simulink model "PhaseII_opalrt_NoProtection"  (Simulink 8.8)
settings: Solver=ode3  StartTime=0.0  StopTime=inf  FixedStep=Ts  RelTol=1e-5  EnableMultiTasking=on
PostLoadFcn:
  | %BESS ctrl
  | Kpf=0.005*3*12;
  | Kif=5*6;
  | 
  | Kpf1=0.005*3*12;
  | Kif1=5*6;
  | Kp_v=0.016*15*35;
  | Ki_v=12*25;
  | 
  | Kp_v1=0.016*15*35;
  | Ki_v1=12*25;
  | 
  | Vabc_B=12.47e3;
  | Vdc_ref=Vabc_B*2;
  | Kpwm=sqrt(2)*Vabc_B/Vdc_ref;
  | ZB=Vabc_B^2/1e6;
  | R=0.005*ZB;
  | Ibasefull=673/2*sqrt(2);
  | 
  | 
  | Ts_Control=1e-4;
  | ts=0.05;
  | delay=0.2;
  | offset=10e3;
  | t_plan=60;
  | t_monitor=.2;
  | t_mon=t_monitor;
  | scalingfactor=1;
  | x=0.5;
  | n=6;
  | %t_plan=1/15;
  | %t_monitor=10/900;
  | %t_mon=10/900;
  | 
  | %t_plan=1/5;
  | %t_monitor=10/300;
  | %t_mon=10/300;
  | %scalingfactor=1/300;
  | 
  | f0=60;
  | 
  | Pabc_B=1e6;
  | Iabc_B=Pabc_B*sqrt(2/3)/Vabc_B;  % pk value
  | Imax_1=2.5;
  | Ptrans_B=Pabc_B*200;
  | 
  | Vdc_ref=Vabc_B*2;
  | 
  | ZB=Vabc_B^2/Pabc_B;
  | L=0.1*ZB/2/pi/60;
  | R=0.1*ZB;
  | C=1/(4*pi^2*(2e3)^2*L);
  | 
  | LL=0.005*ZB/2/pi/60;
  | RR=0.005*ZB;
  | 
  | RC=0.02;
  | 
  | %%% Initial SOC %%%%
  | SOC_ini_BESS1=0.5;
  | ... (+223 lines)
InitFcn:
  | %BESS ctrl
  | Kpf=0.005*3*12;
  | Kif=5*6;
  | 
  | Kpf1=0.005*3*12;
  | Kif1=5*6;
  | Kp_v=0.016*15*35;
  | Ki_v=12*25;
  | 
  | Kp_v1=0.016*15*35;
  | Ki_v1=12*25;
  | 
  | Vabc_B=12.47e3;
  | Vdc_ref=Vabc_B*2;
  | Kpwm=sqrt(2)*Vabc_B/Vdc_ref;
  | ZB=Vabc_B^2/1e6;
  | R=0.005*ZB;
  | Ibasefull=673/2*sqrt(2);
  | 
  | 
  | Ts_Control=1e-4;
  | ts=0.05;
  | delay=0.2;
  | offset=10e3;
  | t_plan=60;
  | t_monitor=.2;
  | t_mon=t_monitor;
  | scalingfactor=1;
  | x=0.5;
  | n=6;
  | %t_plan=1/15;
  | %t_monitor=10/900;
  | %t_mon=10/900;
  | 
  | %t_plan=1/5;
  | %t_monitor=10/300;
  | %t_mon=10/300;
  | %scalingfactor=1/300;
  | 
  | f0=60;
  | 
  | Pabc_B=1e6;
  | Iabc_B=Pabc_B*sqrt(2/3)/Vabc_B;  % pk value
  | Imax_1=2.5;
  | Ptrans_B=Pabc_B*200;
  | 
  | Vdc_ref=Vabc_B*2;
  | 
  | ZB=Vabc_B^2/Pabc_B;
  | L=0.1*ZB/2/pi/60;
  | R=0.1*ZB;
  | C=1/(4*pi^2*(2e3)^2*L);
  | 
  | LL=0.005*ZB/2/pi/60;
  | RR=0.005*ZB;
  | 
  | RC=0.02;
  | 
  | %%% Initial SOC %%%%
  | SOC_ini_BESS1=0.5;
  | ... (+223 lines)
undefined symbols (not defined in the file): D1, Delta, DiscIntNeverNeededParam, Left, PG2ref, type, V
libraries: powerlib x220, powerlib_meascontrol x82, dspstat3 x54, dsparch4 x43, dspswit3 x24, simulink x19, simulink_extras x12, powerlib_extras x11, ssn_lib x7, artemis x6, rtlab x5, rtio_generic_dnp3 x5
(part 2 of 9)

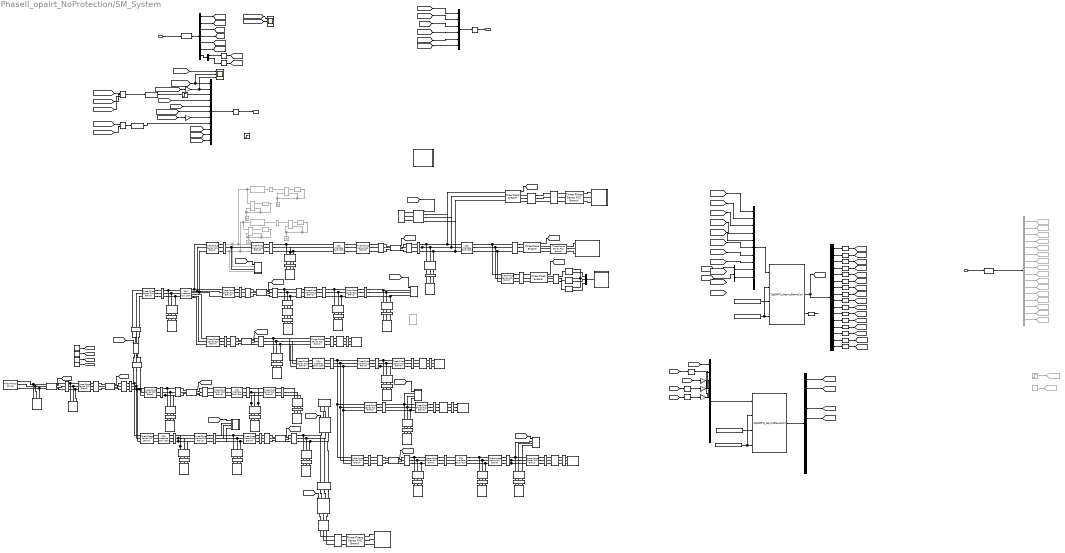
== system PhaseII_opalrt_NoProtection/SM_System ==
  note: DNP3 Communication
  note: Manual Control
  SC2SM : Inport
  SS2SM : Inport  Port=2
  2 kHz1 : dsparch4/Analog Filter Design  method=Butterworth  filttype=Lowpass  N=2  Wlo=2*pi*5  Whi=80  Rp=2  Rs=40
  2 kHz2 : dsparch4/Analog Filter Design  method=Butterworth  filttype=Lowpass  N=2  Wlo=2*pi*5  Whi=80  Rp=2  Rs=40
  2 kHz5 : dsparch4/Analog Filter Design  method=Butterworth  filttype=Lowpass  N=2  Wlo=2*pi*5  Whi=80  Rp=2  Rs=40
  Analog outputs init values1 : Constant  Value=0
  Analog outputs init values2 : Constant  Value=[0 0 0 0 0 0 0 0 0 0 0 0 0 0 0 0 0 0 0 0 0 0 0 0 0 0 0 0 0 0 0 0 0 0 0 0 0 0 0 0 0 0 0 0 0 0 0 0 0 0 0 0 0 0 0 ]
  Analog outputs init values3 : Constant  Value=[0 0 0 0 0 0 0 0 0 0 0 0 0 0 0 0 0 0 0 0 0 0 0 0 0 0 0 0 0 0 0 0 0 0 0 0 0 0 0 0 0 0 0 0 0 0 0 0 0 0 0 0 0 0 0 ]
  Analog outputs init values4 : Constant  Value=0
  Battery 2 : Subsystem  mask{eff=10, area=8e4}
      mask prompts: eff "Efficiency (%)"; area "Area (m^2)"
      mask help: The product of the effeciency, the area covered by the Pv farm and the irradiance in w/m2 will give you the power generate by the PV farm
      mask DialogControl DescGroupVar Prompt: PV farm
      mask DialogControl DescTextVar Prompt: The product of the efficiency, the area covered by the PV farm and the irradiance in W/m2 will give you the power generated by the PV farm.
      mask Display: image(imread('BESS.png'))
  "Battery 1 " : Subsystem  mask{eff=10, area=8e4}
      mask prompts: eff "Efficiency (%)"; area "Area (m^2)"
      mask help: The product of the effeciency, the area covered by the Pv farm and the irradiance in w/m2 will give you the power generate by the PV farm
      mask DialogControl DescGroupVar Prompt: PV farm
      mask DialogControl DescTextVar Prompt: The product of the efficiency, the area covered by the PV farm and the irradiance in W/m2 will give you the power generated by the PV farm.
      mask Display: image(imread('BESS.png'))
  Constant10 : Constant  Value=0.1
  Constant3 : Constant  Commented=on  Value=0.2
  Constant7 : Constant  Value=0.1
  Constant8 : Constant  Value=0.15
  Constant9 : Constant  Value=0.1
  Data Type Conversion{,1..18} (19 alike) : DataTypeConversion
  Demux : Demux  Outputs=3
  Demux13 : Demux  Outputs=16
  Demux14 : Demux  Outputs=10
  Demux17 : Demux  Outputs=2
  Demux2 : Demux  Outputs=[1 3 1 3 1 3 2]
  Demux3 : Demux  Commented=on  Outputs=[1 1 1 1 1 1 1 1 1 1 1 1 1 1 1 1]
  Distribution XFMR 010 : powerlib/Elements/Three-Phase Transformer (Two Windings)  Winding1Connection=Yg  Winding2Connection=Yg  CoreType=Three single-phase transformers  SetSaturation=off  Hysteresis=off  DataFile='hysteresis'  SetInitialFlux=off  Measurements=None  UNITS=pu  NominalPower=[ 750e3 , 60 ]  Winding1=[ 12.47e3 , 0.006*0.5 , 0.004*0.8 ]  Winding2=[ 120*sqrt(3) , 0.006 , 0.004*0.4 ]  Rm=339.61  Lm=332.223  L0=0.5  Saturation=[ 0,0 ; 0.0024,1.2 ; 1.0,1.52 ]  InitialFluxes=[-0.9942658300888 0.50146897071322 0.490639480643619]  MoreParameters=off  BreakLoop=on  DataType=off  TransfoNumber=1
  Distribution XFMR 011 : powerlib/Elements/Three-Phase Transformer (Two Windings)  Winding1Connection=Yg  Winding2Connection=Yg  CoreType=Three single-phase transformers  SetSaturation=off  Hysteresis=off  DataFile='hysteresis'  SetInitialFlux=off  Measurements=None  UNITS=pu  NominalPower=[ 750e3 , 60 ]  Winding1=[ 12.47e3 , 0.003*0.5 , 0.002*0.8 ]  Winding2=[ 120*sqrt(3) , 0.003 , 0.002*0.4 ]  Rm=391.76  Lm=422.949  L0=0.5  Saturation=[ 0,0 ; 0.0024,1.2 ; 1.0,1.52 ]  InitialFluxes=[-0.994208974756347 0.50135973621935 0.490459797609216]  MoreParameters=off  BreakLoop=on  DataType=off  TransfoNumber=1
  Distribution XFMR 012 : powerlib/Elements/Three-Phase Transformer (Two Windings)  Winding1Connection=Yg  Winding2Connection=Yg  CoreType=Three single-phase transformers  SetSaturation=off  Hysteresis=off  DataFile='hysteresis'  SetInitialFlux=off  Measurements=None  UNITS=pu  NominalPower=[ 750e3 , 60 ]  Winding1=[ 12.47e3 , 0.003*0.5 , 0.002*0.8 ]  Winding2=[ 120*sqrt(3) , 0.003 , 0.002*0.4 ]  Rm=391.76  Lm=422.949  L0=0.5  Saturation=[ 0,0 ; 0.0024,1.2 ; 1.0,1.52 ]  InitialFluxes=[-0.994702629209233 0.501353388807825 0.490097029757755]  MoreParameters=off  BreakLoop=on  DataType=off  TransfoNumber=1
  Distribution XFMR 013 : powerlib/Elements/Three-Phase Transformer (Two Windings)  Winding1Connection=Yg  Winding2Connection=Yg  CoreType=Three single-phase transformers  SetSaturation=off  Hysteresis=off  DataFile='hysteresis'  SetInitialFlux=off  Measurements=None  UNITS=pu  NominalPower=[ 750e3 , 60 ]  Winding1=[ 12.47e3 , 0.015*0.5 , 0.01*0.8 ]  Winding2=[ 120*sqrt(3) , 0.015 , 0.01*0.4 ]  Rm=391.76  Lm=422.949  L0=0.5  Saturation=[ 0,0 ; 0.0024,1.2 ; 1.0,1.52 ]  InitialFluxes=[-0.994614702520108 0.501538517038193 0.489928867290745]  MoreParameters=off  BreakLoop=on  DataType=off  TransfoNumber=1
  Distribution XFMR 014 : powerlib/Elements/Three-Phase Transformer (Two Windings)  Winding1Connection=Yg  Winding2Connection=Yg  CoreType=Three single-phase transformers  SetSaturation=off  Hysteresis=off  DataFile='hysteresis'  SetInitialFlux=off  Measurements=None  UNITS=pu  NominalPower=[ 750e3 , 60 ]  Winding1=[ 12.47e3 , 0.003*0.5 , 0.002*0.8 ]  Winding2=[ 120*sqrt(3) , 0.003 , 0.002*0.4 ]  Rm=391.76  Lm=422.949  L0=0.5  Saturation=[ 0,0 ; 0.0024,1.2 ; 1.0,1.52 ]  InitialFluxes=[-0.994115977169703 0.501412072072125 0.48984652002872]  MoreParameters=off  BreakLoop=on  DataType=off  TransfoNumber=1
  Distribution XFMR 02 : powerlib/Elements/Linear Transformer  Commented=on  UNITS=pu  NominalPower=[ 150e3 60 ]  winding1="[ 7.2e3  0.01  0.00667 ]"  winding2="[ 120  0.01  0.00667 ]"  ThreeWindings=off  winding3=[ 315e3 0.002 0.08 ]  RmLm=[ 318.75 327.548 ]  Measurements=None  DataType=off
  Distribution XFMR 03 : powerlib/Elements/Linear Transformer  Commented=on  UNITS=pu  NominalPower=[ 100e3 60 ]  winding1="[ 7.2e3  0.015  0.01 ]"  winding2="[ 120  0.015  0.01 ]"  ThreeWindings=off  winding3=[ 315e3 0.002 0.08 ]  RmLm=[ 308.32 322.496 ]  Measurements=None  DataType=off
  Distribution XFMR 04 : powerlib/Elements/Linear Transformer  Commented=on  UNITS=pu  NominalPower=[ 100e3 60 ]  winding1="[ 7.2e3  0.015  0.01 ]"  winding2="[ 120  0.015  0.01 ]"  ThreeWindings=off  winding3=[ 315e3 0.002 0.08 ]  RmLm=[ 308.32 322.496 ]  Measurements=None  DataType=off
  Distribution XFMR 05 : powerlib/Elements/Linear Transformer  Commented=on  UNITS=pu  NominalPower=[ 100e3 60 ]  winding1="[ 7.2e3  0.015  0.01 ]"  winding2="[ 120  0.015  0.01 ]"  ThreeWindings=off  winding3=[ 315e3 0.002 0.08 ]  RmLm=[ 308.32 322.496 ]  Measurements=None  DataType=off
  Distribution XFMR 06 : powerlib/Elements/Three-Phase Transformer (Two Windings)  Winding1Connection=Yg  Winding2Connection=Yg  CoreType=Three single-phase transformers  SetSaturation=off  Hysteresis=off  DataFile='hysteresis'  SetInitialFlux=off  Measurements=None  UNITS=pu  NominalPower=[ 725e3 , 60 ]  Winding1=[ 12.47e3 , 0.002*0.5 , 0.00133*0.8 ]  Winding2=[ 120*sqrt(3) , 0.002 , 0.00133*0.4 ]  Rm=443.91  Lm=376.523  L0=0.5  Saturation=[ 0,0 ; 0.0024,1.2 ; 1.0,1.52 ]  InitialFluxes=[-0.994629268867217 0.501113638204163 0.49204767683857]  MoreParameters=off  BreakLoop=on  DataType=off  TransfoNumber=1
  Distribution XFMR 07 : powerlib/Elements/Three-Phase Transformer (Two Windings)  Winding1Connection=Yg  Winding2Connection=Yg  CoreType=Three single-phase transformers  SetSaturation=off  Hysteresis=off  DataFile='hysteresis'  SetInitialFlux=off  Measurements=None  UNITS=pu  NominalPower=[ 900e3 , 60 ]  Winding1=[ 12.47e3 , 0.005*0.5 , 0.00333*0.8 ]  Winding2=[ 120*sqrt(3) , 0.005 , 0.00333*0.4 ]  Rm=350.04  Lm=312.414  L0=0.5  Saturation=[ 0,0 ; 0.0024,1.2 ; 1.0,1.52 ]  InitialFluxes=[-0.994045652632512 0.501511608393226 0.490384623138428]  MoreParameters=off  BreakLoop=on  DataType=off  TransfoNumber=1
  Distribution XFMR 08 : powerlib/Elements/Three-Phase Transformer (Two Windings)  Winding1Connection=Yg  Winding2Connection=Yg  CoreType=Three single-phase transformers  SetSaturation=off  Hysteresis=off  DataFile='hysteresis'  SetInitialFlux=off  Measurements=None  UNITS=pu  NominalPower=[ 750e3 , 60 ]  Winding1=[ 12.47e3 , 0.006*0.5 , 0.004*0.8 ]  Winding2=[ 120*sqrt(3) , 0.006 , 0.004*0.4 ]  Rm=339.61  Lm=332.223  L0=0.5  Saturation=[ 0,0 ; 0.0024,1.2 ; 1.0,1.52 ]  InitialFluxes=[-0.993941938198277 0.50151258800202 0.490279152869733]  MoreParameters=off  BreakLoop=on  DataType=off  TransfoNumber=1
  Distribution XFMR 09 : powerlib/Elements/Three-Phase Transformer (Two Windings)  Winding1Connection=Yg  Winding2Connection=Yg  CoreType=Three single-phase transformers  SetSaturation=off  Hysteresis=off  DataFile='hysteresis'  SetInitialFlux=off  Measurements=None  UNITS=pu  NominalPower=[ 750e3 , 60 ]  Winding1=[ 12.47e3 , 0.006*0.5 , 0.004*0.8 ]  Winding2=[ 120*sqrt(3) , 0.006 , 0.004*0.4 ]  Rm=339.61  Lm=332.223  L0=0.5  Saturation=[ 0,0 ; 0.0024,1.2 ; 1.0,1.52 ]  InitialFluxes=[-0.994119371539624 0.501403135186892 0.490542917279175]  MoreParameters=off  BreakLoop=on  DataType=off  TransfoNumber=1
  Distribution XFMR 1 : powerlib/Elements/Three-Phase Transformer (Two Windings)  Winding1Connection=Yg  Winding2Connection=Yg  CoreType=Three single-phase transformers  SetSaturation=off  Hysteresis=off  DataFile='hysteresis'  SetInitialFlux=off  Measurements=None  UNITS=pu  NominalPower=[ 812.5e3 , 60 ]  Winding1=[ 12.47e3 , 0.00089 , 0.00444 ]  Winding2=[ 480 , 0.00089 , 0.00444 ]  Rm=522.135  Lm=557.809  L0=0.5  Saturation=[ 0,0 ; 0.0024,1.2 ; 1.0,1.52 ]  InitialFluxes=[-0.995548930077736 0.501337560469489 0.493145095008447]  MoreParameters=off  BreakLoop=on  DataType=off  TransfoNumber=1
  Distribution XFMR 10 : powerlib/Elements/Three-Phase Transformer (Two Windings)  Winding1Connection=Yg  Winding2Connection=Yg  CoreType=Three single-phase transformers  SetSaturation=off  Hysteresis=off  DataFile='hysteresis'  SetInitialFlux=off  Measurements=None  UNITS=pu  NominalPower=[ 750e3 , 60 ]  Winding1=[ 12.47e3 , 0.00133 , 0.00667 ]  Winding2=[ 480 , 0.00133 , 0.00667 ]  Rm=443.91  Lm=404.751  L0=0.5  Saturation=[ 0,0 ; 0.0024,1.2 ; 1.0,1.52 ]  InitialFluxes=[-0.995768733272171 0.501268557544563 0.49352779195633]  MoreParameters=off  BreakLoop=on  DataType=off  TransfoNumber=1
  Distribution XFMR 11 : powerlib/Elements/Three-Phase Transformer (Two Windings)  Winding1Connection=Yg  Winding2Connection=Yg  CoreType=Three single-phase transformers  SetSaturation=off  Hysteresis=off  DataFile='hysteresis'  SetInitialFlux=off  Measurements=None  UNITS=pu  NominalPower=[ 750e3 , 60 ]  Winding1=[ 12.47e3 , 0.00133 , 0.00667 ]  Winding2=[ 480 , 0.00133 , 0.00667 ]  Rm=443.91  Lm=404.751  L0=0.5  Saturation=[ 0,0 ; 0.0024,1.2 ; 1.0,1.52 ]  InitialFluxes=[-0.994824104245158 0.501648177473995 0.492109909205201]  MoreParameters=off  BreakLoop=on  DataType=off  TransfoNumber=1
  Distribution XFMR 12 : powerlib/Elements/Three-Phase Transformer (Two Windings)  Winding1Connection=Yg  Winding2Connection=Yg  CoreType=Three single-phase transformers  SetSaturation=off  Hysteresis=off  DataFile='hysteresis'  SetInitialFlux=off  Measurements=None  UNITS=pu  NominalPower=[ 750e3 , 60 ]  Winding1=[ 12.47e3 , 0.00133 , 0.00667 ]  Winding2=[ 480 , 0.00133 , 0.00667 ]  Rm=443.91  Lm=404.751  L0=0.5  Saturation=[ 0,0 ; 0.0024,1.2 ; 1.0,1.52 ]  InitialFluxes=[-0.994885331973459 0.501617905967982 0.492199284760507]  MoreParameters=off  BreakLoop=on  DataType=off  TransfoNumber=1
  Distribution XFMR 14 : powerlib/Elements/Three-Phase Transformer (Two Windings)  Winding1Connection=Yg  Winding2Connection=Yg  CoreType=Three single-phase transformers  SetSaturation=off  Hysteresis=off  DataFile='hysteresis'  SetInitialFlux=off  Measurements=None  UNITS=pu  NominalPower=[ 812.5e3 , 60 ]  Winding1=[ 12.47e3 , 0.00089 , 0.00444 ]  Winding2=[ 480 , 0.00089 , 0.00444 ]  Rm=522.135  Lm=557.809  L0=0.5  Saturation=[ 0,0 ; 0.0024,1.2 ; 1.0,1.52 ]  InitialFluxes=[-0.995168363199261 0.501512793303796 0.492597007993423]  MoreParameters=off  BreakLoop=on  DataType=off  TransfoNumber=1
  Distribution XFMR 2 : powerlib/Elements/Three-Phase Transformer (Two Windings)  Winding1Connection=Yg  Winding2Connection=Yg  CoreType=Three single-phase transformers  SetSaturation=off  Hysteresis=off  DataFile='hysteresis'  SetInitialFlux=off  Measurements=None  UNITS=pu  NominalPower=[ 750e3 , 60 ]  Winding1=[ 12.47e3 , 0.00133 , 0.00667 ]  Winding2=[ 480 , 0.00133 , 0.00667 ]  Rm=443.91  Lm=404.751  L0=0.5  Saturation=[ 0,0 ; 0.0024,1.2 ; 1.0,1.52 ]  InitialFluxes=[-0.994824104245158 0.501648177473995 0.492109909205201]  MoreParameters=off  BreakLoop=on  DataType=off  TransfoNumber=1
  Distribution XFMR 3 : powerlib/Elements/Three-Phase Transformer (Two Windings)  Winding1Connection=Yg  Winding2Connection=Yg  CoreType=Three single-phase transformers  SetSaturation=off  Hysteresis=off  DataFile='hysteresis'  SetInitialFlux=off  Measurements=None  UNITS=pu  NominalPower=[ 750e3 , 60 ]  Winding1=[ 12.47e3 , 0.00133 , 0.00667 ]  Winding2=[ 480 , 0.00133 , 0.00667 ]  Rm=443.91  Lm=404.751  L0=0.5  Saturation=[ 0,0 ; 0.0024,1.2 ; 1.0,1.52 ]  InitialFluxes=[-0.995594239290872 0.501339764461854 0.493138938060875]  MoreParameters=off  BreakLoop=on  DataType=off  TransfoNumber=1
  Distribution XFMR 4 : powerlib/Elements/Three-Phase Transformer (Two Windings)  Winding1Connection=Yg  Winding2Connection=Yg  CoreType=Three single-phase transformers  SetSaturation=off  Hysteresis=off  DataFile='hysteresis'  SetInitialFlux=off  Measurements=None  UNITS=pu  NominalPower=[ 750e3 , 60 ]  Winding1=[ 12.47e3 , 0.00133 , 0.00667 ]  Winding2=[ 480 , 0.00133 , 0.00667 ]  Rm=443.91  Lm=404.751  L0=0.5  Saturation=[ 0,0 ; 0.0024,1.2 ; 1.0,1.52 ]  InitialFluxes=[-0.995008547006552 0.501540735777986 0.492046020226542]  MoreParameters=off  BreakLoop=on  DataType=off  TransfoNumber=1
  Distribution XFMR 5 : powerlib/Elements/Three-Phase Transformer (Two Windings)  Winding1Connection=Yg  Winding2Connection=Yg  CoreType=Three single-phase transformers  SetSaturation=off  Hysteresis=off  DataFile='hysteresis'  SetInitialFlux=off  Measurements=None  UNITS=pu  NominalPower=[ 750e3 , 60 ]  Winding1=[ 12.47e3 , 0.00222 , 0.01111 ]  Winding2=[ 480 , 0.00222 , 0.01111 ]  Rm=381.330  Lm=323.959  L0=0.5  Saturation=[ 0,0 ; 0.0024,1.2 ; 1.0,1.52 ]  InitialFluxes=[-0.995775345556504 0.501284393321602 0.493471561656197]  MoreParameters=off  BreakLoop=on  DataType=off  TransfoNumber=1
  Distribution XFMR 6 : powerlib/Elements/Three-Phase Transformer (Two Windings)  Winding1Connection=Yg  Winding2Connection=Yg  CoreType=Three single-phase transformers  SetSaturation=off  Hysteresis=off  DataFile='hysteresis'  SetInitialFlux=off  Measurements=None  UNITS=pu  NominalPower=[ 750e3 , 60 ]  Winding1=[ 12.47e3 , 0.00222 , 0.01111 ]  Winding2=[ 480 , 0.00222 , 0.01111 ]  Rm=381.330  Lm=323.959  L0=0.5  Saturation=[ 0,0 ; 0.0024,1.2 ; 1.0,1.52 ]  InitialFluxes=[-0.995636947856055 0.50134328812622 0.493423111787892]  MoreParameters=off  BreakLoop=on  DataType=off  TransfoNumber=1
  Distribution XFMR 7 : powerlib/Elements/Three-Phase Transformer (Two Windings)  Winding1Connection=Yg  Winding2Connection=Yg  CoreType=Three single-phase transformers  SetSaturation=off  Hysteresis=off  DataFile='hysteresis'  SetInitialFlux=off  Measurements=None  UNITS=pu  NominalPower=[ 750e3 , 60 ]  Winding1=[ 12.47e3 , 0.00111 , 0.00556 ]  Winding2=[ 480 , 0.00111 , 0.00556 ]  Rm=475.200  Lm=495.783  L0=0.5  Saturation=[ 0,0 ; 0.0024,1.2 ; 1.0,1.52 ]  InitialFluxes=[-0.995429112842175 0.501437040144372 0.492976191256826]  MoreParameters=off  BreakLoop=on  DataType=off  TransfoNumber=1
  Distribution XFMR 8 : powerlib/Elements/Three-Phase Transformer (Two Windings)  Winding1Connection=Yg  Winding2Connection=Yg  CoreType=Three single-phase transformers  SetSaturation=off  Hysteresis=off  DataFile='hysteresis'  SetInitialFlux=off  Measurements=None  UNITS=pu  NominalPower=[ 750e3 , 60 ]  Winding1=[ 12.47e3 , 0.00222 , 0.01111 ]  Winding2=[ 480 , 0.00222 , 0.01111 ]  Rm=381.330  Lm=323.959  L0=0.5  Saturation=[ 0,0 ; 0.0024,1.2 ; 1.0,1.52 ]  InitialFluxes=[0.493153694918364 0.501391810391627 -0.995533055661482]  MoreParameters=off  BreakLoop=on  DataType=off  TransfoNumber=1
  Distribution XFMR 9 : powerlib/Elements/Three-Phase Transformer (Two Windings)  Winding1Connection=Yg  Winding2Connection=Yg  CoreType=Three single-phase transformers  SetSaturation=off  Hysteresis=off  DataFile='hysteresis'  SetInitialFlux=off  Measurements=None  UNITS=pu  NominalPower=[ 750e3 , 60 ]  Winding1=[ 12.47e3 , 0.00133 , 0.00667 ]  Winding2=[ 480 , 0.00133 , 0.00667 ]  Rm=443.91  Lm=404.751  L0=0.5  Saturation=[ 0,0 ; 0.0024,1.2 ; 1.0,1.52 ]  InitialFluxes=[-0.995385675641374 0.501454453441104 0.492920662481959]  MoreParameters=off  BreakLoop=on  DataType=off  TransfoNumber=1
  Gain2 : Gain  Gain=Pb/1e6
  Gain3 : Gain
  Gain4 : Gain  Gain=Pb/1e6
  Gain5 : Gain
  Gain6 : Gain  Gain=60
  Gen bus : powerlib/Measurements/Three-Phase V-I Measurement  VoltageMeasurement=phase-to-phase  SetLabelV=on  LabelV=VabcGen  Vpu=off  VpuLL=off  CurrentMeasurement=yes  SetLabelI=on  LabelI=IabcGen  Ipu=off  Pbase=Pb  Vbase=Vb*sqrt(3/2)  OutputType=Complex  PhasorSimulation=off  PSBequivalent=0
  Gen bus1 : powerlib/Measurements/Three-Phase V-I Measurement  VoltageMeasurement=phase-to-phase  SetLabelV=on  LabelV=VabcGen_internal  Vpu=off  VpuLL=off  CurrentMeasurement=yes  SetLabelI=on  LabelI=IabcGen_internal  Ipu=off  Pbase=Pb  Vbase=Vb*sqrt(3/2)  OutputType=Complex  PhasorSimulation=off  PSBequivalent=0
  Generator2 : Subsystem
  Goto1 : Goto  Commented=on  GotoTag=F3  TagVisibility=global
  Goto58 : Goto  Commented=on  GotoTag=S_Y3  TagVisibility=global
  Goto59 : Goto  Commented=on  GotoTag=S_Y4  TagVisibility=global
  Goto66 : Goto  Commented=on  GotoTag=S_Y5  TagVisibility=global
  Goto67 : Goto  Commented=on  GotoTag=S_Y6  TagVisibility=global
  Goto70 : Goto  Commented=on  GotoTag=G1_En  TagVisibility=global
  Goto72 : Goto  Commented=on  GotoTag=Grid_enable  TagVisibility=global
  Goto73 : Goto  Commented=on  GotoTag=S_G1  TagVisibility=global
  Goto74 : Goto  Commented=on  GotoTag=S_Y7  TagVisibility=global
  Goto75 : Goto  Commented=on  GotoTag=S_Y1  TagVisibility=global
  Goto76 : Goto  Commented=on  GotoTag=S_Y2  TagVisibility=global
  Goto77 : Goto  Commented=on  GotoTag=S_G2  TagVisibility=global
  Goto78 : Goto  Commented=on  GotoTag=S_Y8  TagVisibility=global
  Goto79 : Goto  Commented=on  GotoTag=F6  TagVisibility=global
  Goto80 : Goto  Commented=on  GotoTag=F7  TagVisibility=global
  Goto81 : Goto  Commented=on  GotoTag=Manual_Reset  TagVisibility=global
  Goto82 : Goto  Commented=on  GotoTag=Gen_P  TagVisibility=global
  Goto9 : Goto  Commented=on  GotoTag=F5  TagVisibility=global
  Ground{,2..4} (4 alike) : powerlib/Elements/Ground  Commented=on  LConnTagsString=a
  Intellirupter : Subsystem
  Load 1 : powerlib/Elements/Three-Phase Series RLC Load  LConnTagsString=A|B|C  Configuration=Y (grounded)  NominalVoltage=480  Vabc=[ 0.987168 0.986064 0.986504]*277.128  Vabcp=[1e3 1e3 1e3]  NominalFrequency=60  UnbalancedPower=on  ActivePower=10e3  InductivePower=100  CapacitivePower=100  Pabc=[17027.7904 21000.1348 17507.4994]*load_scale  QLabc=[11009.6057 13611.7741 11303.4274]*load_scale/10  QCabc=[0 0 0]  Pabcp=[10e3 9e3 11e3]  QLabcp=[100 90 110]  QCabcp=[100 90 110]  Measurements=None  LoadType=constant PQ
  Load 10 : powerlib/Elements/Three-Phase Series RLC Load  LConnTagsString=A|B|C  Configuration=Y (grounded)  NominalVoltage=480  Vabc=[ 0.994007 0.993686 0.993644]*277.128  Vabcp=[1e3 1e3 1e3]  NominalFrequency=60  UnbalancedPower=on  ActivePower=10e3  InductivePower=100  CapacitivePower=100  Pabc=[39119.69 48245.7642 40221.7746]*load_scale/2  QLabc=[25293.4968 31271.7251 25968.5235]*load_scale/2/10  QCabc=[0 0 0]  Pabcp=[10e3 9e3 11e3]  QLabcp=[100 90 110]  QCabcp=[100 90 110]  Measurements=None  LoadType=constant PQ
  Load 11 : powerlib/Elements/Three-Phase Series RLC Load  LConnTagsString=A|B|C  Configuration=Y (grounded)  NominalVoltage=480  Vabc=[ 0.992968 0.992478 0.992611]*277.128  Vabcp=[1e3 1e3 1e3]  NominalFrequency=60  UnbalancedPower=on  ActivePower=10e3  InductivePower=100  CapacitivePower=100  Pabc=[46970.1648 57927.6445 48293.4139]*load_scale  QLabc=[30369.354 37547.2833 31179.8439]*load_scale/10  QCabc=[0 0 0]  Pabcp=[10e3 9e3 11e3]  QLabcp=[100 90 110]  QCabcp=[100 90 110]  Measurements=None  LoadType=constant PQ
  Load 12 : powerlib/Elements/Three-Phase Series RLC Load  LConnTagsString=A|B|C  Configuration=Y (grounded)  NominalVoltage=480  Vabc=[ 0.993588 0.993244 0.993249]*277.128  Vabcp=[1e3 1e3 1e3]  NominalFrequency=60  UnbalancedPower=on  ActivePower=10e3  InductivePower=100  CapacitivePower=100  Pabc=[40129.5633 49491.2267 41260.0981]*load_scale  QLabc=[25946.4474 32079.0035 26638.8999]*load_scale/10  QCabc=[0 0 0]  Pabcp=[10e3 9e3 11e3]  QLabcp=[100 90 110]  QCabcp=[100 90 110]  Measurements=None  LoadType=constant PQ
  Load 13 : powerlib/Elements/Three-Phase Series RLC Load  LConnTagsString=A|B|C  Configuration=Y (grounded)  NominalVoltage=480  Vabc=[ 0.992901 0.992425 0.992496]*277.128  Vabcp=[1e3 1e3 1e3]  NominalFrequency=60  UnbalancedPower=on  ActivePower=10e3  InductivePower=100  CapacitivePower=100  Pabc=[1 1 1]  QLabc=[0 0 0]  QCabc=[0 0 0]  Pabcp=[10e3 9e3 11e3]  QLabcp=[100 90 110]  QCabcp=[100 90 110]  Measurements=None  LoadType=constant PQ
  Load 14 : powerlib/Elements/Three-Phase Series RLC Load  LConnTagsString=A|B|C  Configuration=Y (grounded)  NominalVoltage=480  Vabc=[ 0.992968 0.992478 0.992611]*277.128  Vabcp=[1e3 1e3 1e3]  NominalFrequency=60  UnbalancedPower=on  ActivePower=10e3  InductivePower=100  CapacitivePower=100  Pabc=[46970.1648 57927.6445 48293.4139]*load_scale  QLabc=[30369.354 37547.2833 31179.8439]*load_scale/10  QCabc=[0 0 0]  Pabcp=[10e3 9e3 11e3]  QLabcp=[100 90 110]  QCabcp=[100 90 110]  Measurements=None  LoadType=constant PQ
  Load 15 : powerlib/Elements/Three-Phase Series RLC Load  LConnTagsString=A|B|C  Configuration=Y (grounded)  NominalVoltage=480  Vabc=[ 0.992901 0.992425 0.992496]*277.128  Vabcp=[1e3 1e3 1e3]  NominalFrequency=60  UnbalancedPower=on  ActivePower=10e3  InductivePower=100  CapacitivePower=100  Pabc=[1 1 1]  QLabc=[0 0 0]  QCabc=[0 0 0]  Pabcp=[10e3 9e3 11e3]  QLabcp=[100 90 110]  QCabcp=[100 90 110]  Measurements=None  LoadType=constant PQ
  Load 2 : powerlib/Elements/Three-Phase Series RLC Load  LConnTagsString=A|B|C  Configuration=Y (grounded)  NominalVoltage=480  Vabc=[ 0.994058 0.994595 0.993585]*277.128  Vabcp=[1e3 1e3 1e3]  NominalFrequency=60  UnbalancedPower=on  ActivePower=10e3  InductivePower=100  CapacitivePower=100  Pabc=[81043.4347 89864.2131 82168.4451]*load_scale  QLabc=[52061.1336 58247.7865 53085.0614]*load_scale/10  QCabc=[0 0 0]  Pabcp=[10e3 9e3 11e3]  QLabcp=[100 90 110]  QCabcp=[100 90 110]  Measurements=None  LoadType=constant PQ
  Load 3 : powerlib/Elements/Three-Phase Series RLC Load  LConnTagsString=A|B|C  Configuration=Y (grounded)  NominalVoltage=480  Vabc=[ 0.992901 0.992425 0.992496]*277.128  Vabcp=[1e3 1e3 1e3]  NominalFrequency=60  UnbalancedPower=on  ActivePower=10e3  InductivePower=100  CapacitivePower=100  Pabc=[49962.928 61618.5773 51370.4895]*load_scale/2  QLabc=[32304.3756 39939.6557 33166.5069]*load_scale/2/10  QCabc=[0 0 0]  Pabcp=[10e3 9e3 11e3]  QLabcp=[100 90 110]  QCabcp=[100 90 110]  Measurements=None  LoadType=constant PQ
  Load 4 : powerlib/Elements/Three-Phase Series RLC Load  LConnTagsString=A|B|C  Configuration=Y (grounded)  NominalVoltage=480  Vabc=[ 0.99408 0.993727 0.99369]*277.128  Vabcp=[1e3 1e3 1e3]  NominalFrequency=60  UnbalancedPower=on  ActivePower=10e3  InductivePower=100  CapacitivePower=100  Pabc=[35013.8548 43182.0953 36000.2693]*load_scale/2  QLabc=[22638.7997 27989.5787 23242.9784]*load_scale/10  QCabc=[0 0 0]  Pabcp=[10e3 9e3 11e3]  QLabcp=[100 90 110]  QCabcp=[100 90 110]  Measurements=None  LoadType=constant PQ
  Load 5 : powerlib/Elements/Three-Phase Series RLC Load  LConnTagsString=A|B|C  Configuration=Y (grounded)  NominalVoltage=480  Vabc=[ 0.990244 0.989037 0.989784]*277.128  Vabcp=[1e3 1e3 1e3]  NominalFrequency=60  UnbalancedPower=on  ActivePower=10e3  InductivePower=100  CapacitivePower=100  Pabc=[28836.6737 35563.8646 29649.0639]*load_scale/2  QLabc=[18644.8388 23051.6278 19142.4277]*load_scale/2/10  QCabc=[0 0 0]  Pabcp=[10e3 9e3 11e3]  QLabcp=[100 90 110]  QCabcp=[100 90 110]  Measurements=None  LoadType=constant PQ
  Load 6 : powerlib/Elements/Three-Phase Series RLC Load  LConnTagsString=A|B|C  Configuration=Y (grounded)  NominalVoltage=480  Vabc=[ 0.989951 0.988653 0.989471]*277.128  Vabcp=[1e3 1e3 1e3]  NominalFrequency=60  UnbalancedPower=on  ActivePower=10e3  InductivePower=100  CapacitivePower=100  Pabc=[29787.5763 36736.5994 30626.7554]*load_scale/2  QLabc=[19259.6609 23811.7658 19773.6581]*load_scale/2/10  QCabc=[0 0 0]  Pabcp=[10e3 9e3 11e3]  QLabcp=[100 90 110]  QCabcp=[100 90 110]  Measurements=None  LoadType=constant PQ
  Load 7 : powerlib/Elements/Three-Phase Series RLC Load  LConnTagsString=A|B|C  Configuration=Y (grounded)  NominalVoltage=480  Vabc=[ 0.993519 0.993097 0.993157]*277.128  Vabcp=[1e3 1e3 1e3]  NominalFrequency=60  UnbalancedPower=on  ActivePower=10e3  InductivePower=100  CapacitivePower=100  Pabc=[64484.4635 79527.7832 66301.1275]*load_scale  QLabc=[41693.5199 51547.9652 42806.2264]*load_scale/10  QCabc=[0 0 0]  Pabcp=[10e3 9e3 11e3]  QLabcp=[100 90 110]  QCabcp=[100 90 110]  Measurements=None  LoadType=constant PQ
  Load 8 : powerlib/Elements/Three-Phase Series RLC Load  LConnTagsString=A|B|C  Configuration=Y (grounded)  NominalVoltage=480  Vabc=[ 0.991121 0.990439 0.991202]*277.128  Vabcp=[1e3 1e3 1e3]  NominalFrequency=60  UnbalancedPower=on  ActivePower=10e3  InductivePower=100  CapacitivePower=100  Pabc=[24399.1283 30091.1022 25086.5034]*load_scale  QLabc=[15775.6688 19504.317 16196.686]*load_scale/10  QCabc=[0 0 0]  Pabcp=[10e3 9e3 11e3]  QLabcp=[100 90 110]  QCabcp=[100 90 110]  Measurements=None  LoadType=constant PQ
  Load 9 : powerlib/Elements/Three-Phase Series RLC Load  LConnTagsString=A|B|C  Configuration=Y (grounded)  NominalVoltage=480  Vabc=[ 0.992758 0.992152 0.992379]*277.128  Vabcp=[1e3 1e3 1e3]  NominalFrequency=60  UnbalancedPower=on  ActivePower=10e3  InductivePower=100  CapacitivePower=100  Pabc=[52815.6357 65136.7817 54303.5641]*load_scale  QLabc=[34148.842 42220.0698 35060.198]*load_scale/10  QCabc=[0 0 0]  Pabcp=[10e3 9e3 11e3]  QLabcp=[100 90 110]  QCabcp=[100 90 110]  Measurements=None  LoadType=constant PQ
  Load Flow Bus : powerlib/Measurements/Load Flow Bus  LConnTagsString=a|b|c  RConnTagsString=a|b|c  Phases=ABC  Connectors=on both sides  ID=BUS_1  Vbase=7.2e3  Vref=[1 1 1]  Vangle=[0 -120 120]  VLF=1  VLFb=1  VLFc=1  angleLF=0  angleLFb=-120  angleLFc=120
  Load Flow Bus20 : powerlib/Measurements/Load Flow Bus  LConnTagsString=a|b|c  RConnTagsString=a|b|c  Phases=ABC  Connectors=on both sides  ID=BUS_2  Vbase=7.2e3  Vref=[1 1 1]  Vangle=[0 -120 120]  VLF=0.9976  VLFb=0.9981  VLFc=0.9973  angleLF=-0.1269  angleLFb=-120.1  angleLFc=119.9
  Load Flow Bus21 : powerlib/Measurements/Load Flow Bus  LConnTagsString=a|b|c  RConnTagsString=a|b|c  Phases=ABC  Connectors=on both sides  ID=BUS_11  Vbase=7.2e3  Vref=[1 1 1]  Vangle=[0 -120 120]  VLF=0.9972  VLFb=0.9977  VLFc=0.997  angleLF=-0.1433  angleLFb=-120.1  angleLFc=119.9
  Load Flow Bus22 : powerlib/Measurements/Load Flow Bus  LConnTagsString=a|b|c  RConnTagsString=a|b|c  Phases=ABC  Connectors=on both sides  ID=BUS_12  Vbase=7.2e3  Vref=[1 1 1]  Vangle=[0 -120 120]  VLF=0.9972  VLFb=0.9977  VLFc=0.997  angleLF=-0.1436  angleLFb=-120.1  angleLFc=119.9
  Load Flow Bus23 : powerlib/Measurements/Load Flow Bus  LConnTagsString=a|b|c  RConnTagsString=a|b|c  Phases=ABC  Connectors=on both sides  ID=BUS_3_0  Vbase=480/sqrt(3)  Vref=[1 1 1]  Vangle=[0 -120 120]  VLF=0.9935  VLFb=0.9931  VLFc=0.9932  angleLF=-0.3687  angleLFb=-120.4  angleLFc=119.6
  Load Flow Bus24 : powerlib/Measurements/Load Flow Bus  LConnTagsString=a|b|c  RConnTagsString=a|b|c  Phases=ABC  Connectors=on both sides  ID=BUS_4_0  Vbase=480/sqrt(3)  Vref=[1 1 1]  Vangle=[0 -120 120]  VLF=0.9911  VLFb=0.9904  VLFc=0.9912  angleLF=119.5  angleLFb=-120.6  angleLFc=-0.5043
  Load Flow Bus25 : powerlib/Measurements/Load Flow Bus  LConnTagsString=a|b|c  RConnTagsString=a|b|c  Phases=ABC  Connectors=on both sides  ID=BUS_5_0  Vbase=480/sqrt(3)  Vref=[1 1 1]  Vangle=[0 -120 120]  VLF=0.9928  VLFb=0.9922  VLFc=0.9924  angleLF=-0.413  angleLFb=-120.5  angleLFc=119.6
  Load Flow Bus26 : powerlib/Measurements/Load Flow Bus  LConnTagsString=a|b|c  RConnTagsString=a|b|c  Phases=ABC  Connectors=on both sides  ID=BUS_6_0  Vbase=480/sqrt(3)  Vref=[1 1 1]  Vangle=[0 -120 120]  VLF=0.9902  VLFb=0.989  VLFc=0.9898  angleLF=-0.5603  angleLFb=-120.6  angleLFc=119.4
  Load Flow Bus27 : powerlib/Measurements/Load Flow Bus  LConnTagsString=a|b|c  RConnTagsString=a|b|c  Phases=ABC  Connectors=on both sides  ID=BUS_7_0  Vbase=480/sqrt(3)  Vref=[1 1 1]  Vangle=[0 -120 120]  VLF=0.994  VLFb=0.9937  VLFc=0.9936  angleLF=-0.3395  angleLFb=-120.4  angleLFc=119.7
  Load Flow Bus28 : powerlib/Measurements/Load Flow Bus  LConnTagsString=a|b|c  RConnTagsString=a|b|c  Phases=ABC  Connectors=on both sides  ID=BUS_8_0  Vbase=480/sqrt(3)  Vref=[1 1 1]  Vangle=[0 -120 120]  VLF=0.99  VLFb=0.9887  VLFc=0.9895  angleLF=-0.5766  angleLFb=-120.7  angleLFc=119.4
  Load Flow Bus29 : powerlib/Measurements/Load Flow Bus  LConnTagsString=a|b|c  RConnTagsString=a|b|c  Phases=ABC  Connectors=on both sides  ID=BUS_9_0  Vbase=480/sqrt(3)  Vref=[1 1 1]  Vangle=[0 -120 120]  VLF=0.9929  VLFb=0.9924  VLFc=0.9925  angleLF=-0.4047  angleLFb=-120.4  angleLFc=119.6
  Load Flow Bus30 : powerlib/Measurements/Load Flow Bus  LConnTagsString=a|b|c  RConnTagsString=a|b|c  Phases=ABC  Connectors=on both sides  ID=BUS_10_0  Vbase=120  Vref=[1 1 1]  Vangle=[0 -120 120]  VLF=0.9855  VLFb=0.9834  VLFc=0.985  angleLF=-0.08438  angleLFb=-120  angleLFc=119.9
  Load Flow Bus31 : powerlib/Measurements/Load Flow Bus  LConnTagsString=a|b|c  RConnTagsString=a|b|c  Phases=ABC  Connectors=on both sides  ID=BUS_3  Vbase=7.2e3  Vref=[1 1 1]  Vangle=[0 -120 120]  VLF=0.9976  VLFb=0.9981  VLFc=0.9973  angleLF=-0.1275  angleLFb=-120.1  angleLFc=119.9
  Load Flow Bus32 : powerlib/Measurements/Load Flow Bus  LConnTagsString=a|b|c  RConnTagsString=a|b|c  Phases=ABC  Connectors=on both sides  ID=BUS_11_0  Vbase=480/sqrt(3)  Vref=[1 1 1]  Vangle=[0 -120 120]  VLF=0.993  VLFb=0.9925  VLFc=0.9926  angleLF=-0.3966  angleLFb=-120.4  angleLFc=119.6
  Load Flow Bus33 : powerlib/Measurements/Load Flow Bus  LConnTagsString=a|b|c  RConnTagsString=a|b|c  Phases=ABC  Connectors=on both sides  ID=BUS_12_0  Vbase=480/sqrt(3)  Vref=[1 1 1]  Vangle=[0 -120 120]  VLF=0.9936  VLFb=0.9932  VLFc=0.9932  angleLF=-0.3599  angleLFb=-120.4  angleLFc=119.6
  Load Flow Bus36 : powerlib/Measurements/Load Flow Bus  LConnTagsString=a|b|c  RConnTagsString=a|b|c  Phases=ABC  Connectors=on both sides  ID=BUS_13  Vbase=7.2e3  Vref=[1 1 1]  Vangle=[0 -120 120]  VLF=0.997  VLFb=0.9982  VLFc=0.9966  angleLF=-0.1665  angleLFb=-120.1  angleLFc=119.9
  Load Flow Bus37 : powerlib/Measurements/Load Flow Bus  LConnTagsString=a|b|c  RConnTagsString=a|b|c  Phases=ABC  Connectors=on both sides  ID=BUS_14  Vbase=7.2e3  Vref=[1 1 1]  Vangle=[0 -120 120]  VLF=0.997  VLFb=0.9982  VLFc=0.9966  angleLF=-0.1669  angleLFb=-120.1  angleLFc=119.9
  Load Flow Bus38 : powerlib/Measurements/Load Flow Bus  LConnTagsString=a|b|c  RConnTagsString=a|b|c  Phases=ABC  Connectors=on both sides  ID=BUS_15  Vbase=7.2e3  Vref=[1 1 1]  Vangle=[0 -120 120]  VLF=0.9969  VLFb=0.9982  VLFc=0.9966  angleLF=-0.167  angleLFb=-120.1  angleLFc=119.9
  Load Flow Bus39 : powerlib/Measurements/Load Flow Bus  LConnTagsString=a|b|c  RConnTagsString=a|b|c  Phases=ABC  Connectors=on both sides  ID=BUS_14_0  Vbase=480/sqrt(3)  Vref=[1 1 1]  Vangle=[0 -120 120]  VLF=0.9941  VLFb=0.9946  VLFc=0.9936  angleLF=-0.341  angleLFb=-120.3  angleLFc=119.7
  Load Flow Bus40 : powerlib/Measurements/Load Flow Bus  LConnTagsString=a|b|c  RConnTagsString=a|b|c  Phases=ABC  Connectors=on both sides  ID=BUS_15_0  Vbase=480/sqrt(3)  Vref=[1 1 1]  Vangle=[0 -120 120]  VLF=0.9872  VLFb=0.9861  VLFc=0.9865  angleLF=-0.746  angleLFb=-120.8  angleLFc=119.3
  Load Flow Bus41 : powerlib/Measurements/Load Flow Bus  Commented=on  LConnTagsString=a  RConnTagsString=a  Phases=A  Connectors=on both sides  ID=BUS_27  Vbase=7.2e3  Vref=1  Vangle=0  VLF=0.9964  VLFb=NaN  VLFc=NaN  angleLF=-0.1708  angleLFb=NaN  angleLFc=NaN
  Load Flow Bus42 : powerlib/Measurements/Load Flow Bus  Commented=on  LConnTagsString=a  RConnTagsString=a  Phases=C  Connectors=on both sides  ID=BUS_28  Vbase=7.2e3  Vref=1  Vangle=120  VLF=NaN  VLFb=NaN  VLFc=0.9958  angleLF=NaN  angleLFb=NaN  angleLFc=119.9
      settings: AttributesFormatString=|
      | %<ID>
      | %<Vbase>V
      | %<VLFc>pu
      | %<angleLFc>deg.
  Load Flow Bus43 : powerlib/Measurements/Load Flow Bus  LConnTagsString=a|b|c  RConnTagsString=a|b|c  Phases=ABC  Connectors=on both sides  ID=BUS_16  Vbase=7.2e3  Vref=[1 1 1]  Vangle=[0 -120 120]  VLF=0.9972  VLFb=0.9976  VLFc=0.9969  angleLF=-0.1422  angleLFb=-120.1  angleLFc=119.9
  Load Flow Bus44 : powerlib/Measurements/Load Flow Bus  LConnTagsString=a|b|c  RConnTagsString=a|b|c  Phases=ABC  Connectors=on both sides  ID=BUS_4  Vbase=7.2e3  Vref=[1 1 1]  Vangle=[0 -120 120]  VLF=0.9975  VLFb=0.9981  VLFc=0.9973  angleLF=-0.1279  angleLFb=-120.1  angleLFc=119.9
  Load Flow Bus45 : powerlib/Measurements/Load Flow Bus  LConnTagsString=a|b|c  RConnTagsString=a|b|c  Phases=ABC  Connectors=on both sides  ID=BUS_16_0  Vbase=480/sqrt(3)  Vref=[1 1 1]  Vangle=[0 -120 120]  VLF=0.9941  VLFb=0.9937  VLFc=0.9937  angleLF=-0.331  angleLFb=-120.4  angleLFc=119.7
  Load Flow Bus46 : powerlib/Measurements/Load Flow Bus  LConnTagsString=a|b|c  RConnTagsString=a|b|c  Phases=ABC  Connectors=on both sides  ID=BUS_17  Vbase=7.2e3  Vref=[1 1 1]  Vangle=[0 -120 120]  VLF=0.9972  VLFb=0.9975  VLFc=0.9969  angleLF=-0.1447  angleLFb=-120.1  angleLFc=119.9
  Load Flow Bus47 : powerlib/Measurements/Load Flow Bus  LConnTagsString=a|b|c  RConnTagsString=a|b|c  Phases=ABC  Connectors=on both sides  ID=BUS_17_0  Vbase=120  Vref=[1 1 1]  Vangle=[0 -120 120]  VLF=0.9957  VLFb=0.9958  VLFc=0.9954  angleLF=-0.1373  angleLFb=-120.1  angleLFc=119.9
  Load Flow Bus48 : powerlib/Measurements/Load Flow Bus  LConnTagsString=a|b|c  RConnTagsString=a|b|c  Phases=ABC  Connectors=on both sides  ID=BUS_18  Vbase=7.2e3  Vref=[1 1 1]  Vangle=[0 -120 120]  VLF=0.997  VLFb=0.997  VLFc=0.9966  angleLF=-0.151  angleLFb=-120.2  angleLFc=119.8
  Load Flow Bus49 : powerlib/Measurements/Load Flow Bus  LConnTagsString=a|b|c  RConnTagsString=a|b|c  Phases=ABC  Connectors=on both sides  ID=BUS_19  Vbase=7.2e3  Vref=[1 1 1]  Vangle=[0 -120 120]  VLF=0.9968  VLFb=0.9968  VLFc=0.9965  angleLF=-0.1562  angleLFb=-120.2  angleLFc=119.8
  Load Flow Bus50 : powerlib/Measurements/Load Flow Bus  LConnTagsString=a|b|c  RConnTagsString=a|b|c  Phases=ABC  Connectors=on both sides  ID=BUS_20  Vbase=7.2e3  Vref=[1 1 1]  Vangle=[0 -120 120]  VLF=0.9968  VLFb=0.9968  VLFc=0.9965  angleLF=-0.157  angleLFb=-120.2  angleLFc=119.8
  Load Flow Bus51 : powerlib/Measurements/Load Flow Bus  LConnTagsString=a|b|c  RConnTagsString=a|b|c  Phases=ABC  Connectors=on both sides  ID=BUS_19_0  Vbase=120  Vref=[1 1 1]  Vangle=[0 -120 120]  VLF=0.9931  VLFb=0.9923  VLFc=0.9927  angleLF=-0.138  angleLFb=-120.1  angleLFc=119.8
  Load Flow Bus52 : powerlib/Measurements/Load Flow Bus  LConnTagsString=a|b|c  RConnTagsString=a|b|c  Phases=ABC  Connectors=on both sides  ID=BUS_20_0  Vbase=120  Vref=[1 1 1]  Vangle=[0 -120 120]  VLF=0.9926  VLFb=0.9916  VLFc=0.9922  angleLF=-0.1366  angleLFb=-120.1  angleLFc=119.8
  Load Flow Bus53 : powerlib/Measurements/Load Flow Bus  LConnTagsString=a|b|c  RConnTagsString=a|b|c  Phases=ABC  Connectors=on both sides  ID=BUS_21  Vbase=7.2e3  Vref=[1 1 1]  Vangle=[0 -120 120]  VLF=0.9969  VLFb=0.9969  VLFc=0.9965  angleLF=-0.1533  angleLFb=-120.2  angleLFc=119.8
  Load Flow Bus54 : powerlib/Measurements/Load Flow Bus  LConnTagsString=a|b|c  RConnTagsString=a|b|c  Phases=ABC  Connectors=on both sides  ID=BUS_22  Vbase=7.2e3  Vref=[1 1 1]  Vangle=[0 -120 120]  VLF=0.9969  VLFb=0.9969  VLFc=0.9965  angleLF=-0.1535  angleLFb=-120.2  angleLFc=119.8
  Load Flow Bus55 : powerlib/Measurements/Load Flow Bus  LConnTagsString=a|b|c  RConnTagsString=a|b|c  Phases=ABC  Connectors=on both sides  ID=BUS_5  Vbase=7.2e3  Vref=[1 1 1]  Vangle=[0 -120 120]  VLF=0.9975  VLFb=0.9981  VLFc=0.9973  angleLF=-0.1283  angleLFb=-120.1  angleLFc=119.9
  Load Flow Bus56 : powerlib/Measurements/Load Flow Bus  LConnTagsString=a|b|c  RConnTagsString=a|b|c  Phases=ABC  Connectors=on both sides  ID=BUS_21_0  Vbase=120  Vref=[1 1 1]  Vangle=[0 -120 120]  VLF=0.9921  VLFb=0.991  VLFc=0.9916  angleLF=-0.13  angleLFb=-120.1  angleLFc=119.9
  Load Flow Bus57 : powerlib/Measurements/Load Flow Bus  LConnTagsString=a|b|c  RConnTagsString=a|b|c  Phases=ABC  Connectors=on both sides  ID=BUS_22_0  Vbase=120  Vref=[1 1 1]  Vangle=[0 -120 120]  VLF=0.9937  VLFb=0.9929  VLFc=0.9932  angleLF=-0.1379  angleLFb=-120.1  angleLFc=119.8
  Load Flow Bus58 : powerlib/Measurements/Load Flow Bus  LConnTagsString=a|b|c  RConnTagsString=a|b|c  Phases=ABC  Connectors=on both sides  ID=BUS_23  Vbase=7.2e3  Vref=[1 1 1]  Vangle=[0 -120 120]  VLF=0.9969  VLFb=0.9969  VLFc=0.9965  angleLF=-0.1517  angleLFb=-120.2  angleLFc=119.8
  Load Flow Bus59 : powerlib/Measurements/Load Flow Bus  LConnTagsString=a|b|c  RConnTagsString=a|b|c  Phases=ABC  Connectors=on both sides  ID=BUS_24  Vbase=7.2e3  Vref=[1 1 1]  Vangle=[0 -120 120]  VLF=0.9969  VLFb=0.9967  VLFc=0.9965  angleLF=-0.1513  angleLFb=-120.2  angleLFc=119.8
  Load Flow Bus60 : powerlib/Measurements/Load Flow Bus  LConnTagsString=a|b|c  RConnTagsString=a|b|c  Phases=ABC  Connectors=on both sides  ID=BUS_25  Vbase=7.2e3  Vref=[1 1 1]  Vangle=[0 -120 120]  VLF=0.9969  VLFb=0.9967  VLFc=0.9964  angleLF=-0.1528  angleLFb=-120.2  angleLFc=119.8
  Load Flow Bus61 : powerlib/Measurements/Load Flow Bus  LConnTagsString=a|b|c  RConnTagsString=a|b|c  Phases=ABC  Connectors=on both sides  ID=BUS_26  Vbase=7.2e3  Vref=[1 1 1]  Vangle=[0 -120 120]  VLF=0.9969  VLFb=0.9966  VLFc=0.9964  angleLF=-0.1542  angleLFb=-120.2  angleLFc=119.8
  Load Flow Bus62 : powerlib/Measurements/Load Flow Bus  LConnTagsString=a|b|c  RConnTagsString=a|b|c  Phases=ABC  Connectors=on both sides  ID=BUS_23_0  Vbase=120  Vref=[1 1 1]  Vangle=[0 -120 120]  VLF=0.9946  VLFb=0.994  VLFc=0.9941  angleLF=-0.1402  angleLFb=-120.1  angleLFc=119.8
  Load Flow Bus63 : powerlib/Measurements/Load Flow Bus  LConnTagsString=a|b|c  RConnTagsString=a|b|c  Phases=ABC  Connectors=on both sides  ID=BUS_24_0  Vbase=120  Vref=[1 1 1]  Vangle=[0 -120 120]  VLF=0  VLFb=0.9941  VLFc=0.9943  angleLF=0  angleLFb=-120.1  angleLFc=119.8
  Load Flow Bus64 : powerlib/Measurements/Load Flow Bus  LConnTagsString=a|b|c  RConnTagsString=a|b|c  Phases=ABC  Connectors=on both sides  ID=BUS_25_0  Vbase=120  Vref=[1 1 1]  Vangle=[0 -120 120]  VLF=0  VLFb=0  VLFc=0.9857  angleLF=0  angleLFb=0  angleLFc=119.9
  Load Flow Bus65 : powerlib/Measurements/Load Flow Bus  LConnTagsString=a|b|c  RConnTagsString=a|b|c  Phases=ABC  Connectors=on both sides  ID=BUS_26_0  Vbase=120  Vref=[1 1 1]  Vangle=[0 -120 120]  VLF=0.9949  VLFb=0.9942  VLFc=0.9944  angleLF=-0.1445  angleLFb=-120.2  angleLFc=119.8
  Load Flow Bus66 : powerlib/Measurements/Load Flow Bus  LConnTagsString=a|b|c  RConnTagsString=a|b|c  Phases=ABC  Connectors=on both sides  ID=BUS_6  Vbase=7.2e3  Vref=[1 1 1]  Vangle=[0 -120 120]  VLF=0.9976  VLFb=0.9981  VLFc=0.9973  angleLF=-0.1275  angleLFb=-120.1  angleLFc=119.9
  Load Flow Bus67 : powerlib/Measurements/Load Flow Bus  LConnTagsString=a|b|c  RConnTagsString=a|b|c  Phases=ABC  Connectors=on both sides  ID=BUS_7  Vbase=7.2e3  Vref=[1 1 1]  Vangle=[0 -120 120]  VLF=0.9975  VLFb=0.998  VLFc=0.9973  angleLF=-0.1287  angleLFb=-120.1  angleLFc=119.9
  Load Flow Bus68 : powerlib/Measurements/Load Flow Bus  LConnTagsString=a|b|c  RConnTagsString=a|b|c  Phases=ABC  Connectors=on both sides  ID=BUS_8  Vbase=7.2e3  Vref=[1 1 1]  Vangle=[0 -120 120]  VLF=0.9975  VLFb=0.998  VLFc=0.9972  angleLF=-0.1295  angleLFb=-120.1  angleLFc=119.9
  Load Flow Bus69 : powerlib/Measurements/Load Flow Bus  LConnTagsString=a|b|c  RConnTagsString=a|b|c  Phases=ABC  Connectors=on both sides  ID=BUS_9  Vbase=7.2e3  Vref=[1 1 1]  Vangle=[0 -120 120]  VLF=0.9974  VLFb=0.998  VLFc=0.9971  angleLF=-0.1354  angleLFb=-120.1  angleLFc=119.9
  Load Flow Bus70 : powerlib/Measurements/Load Flow Bus  LConnTagsString=a|b|c  RConnTagsString=a|b|c  Phases=ABC  Connectors=on both sides  ID=BUS_10  Vbase=7.2e3  Vref=[1 1 1]  Vangle=[0 -120 120]  VLF=0.9973  VLFb=0.9978  VLFc=0.997  angleLF=-0.1412  angleLFb=-120.1  angleLFc=119.9
  Logical Operator : Logic  Operator=NOT  AllPortsSameDT=off  OutDataTypeStr=boolean
  Logical Operator1 : Logic  Inputs=3  AllPortsSameDT=off  OutDataTypeStr=boolean
  Logical Operator2 : Logic  Operator=NOT  AllPortsSameDT=off  OutDataTypeStr=boolean
  Logical Operator8 : Logic  AllPortsSameDT=off  OutDataTypeStr=boolean
  Memory : Memory
  Memory1 : Memory
  Mux1 : Mux  Inputs=[3 3 1 3 3 3 3 1 1 1 1]
  Mux13 : Mux  Inputs=[1 1 1 1 1 1 1 1 1 1]
  Mux16 : Mux  Inputs=[1 14]
  Mux17 : Mux  Inputs=[1 14]
  Mux2 : Mux  Inputs=[3 3 1 3 3 3]
  Mux3 : Mux  Inputs=[15 15 15 15 15 15 15 15 15 15 15]
  OpComm1 : rtlab/OpComm  nbport=1  groupe_acq=1  subsys_rate=Ts  st=Ts  Synchronization=on  Interpolation=on  Threshold=1.0  Missed_Data=off  Sim_Time=off  Samples=off  dynSigOut=off  from_console=1  warning_done=off  writeOpCommFile=off  Offset=off
  OpComm2 : rtlab/OpComm  nbport=1  groupe_acq=1  subsys_rate=Ts  st=Ts  Synchronization=on  Interpolation=on  Threshold=1.0  Missed_Data=off  Sim_Time=off  Samples=off  dynSigOut=off  from_console=0  warning_done=off  writeOpCommFile=off  Offset=off
  OpDNP3_AsyncSlaveCtrl : rtio_generic_dnp3/OpDNP3_AsyncSlaveCtrl  dev_id=1  nbr_aout=16  nbr_bout=1  cfg_name='AsyncDNP3_Slave_cfg.xml'  exe_name='AsyncDNP3_Slave'  nic_name='eth3'  link_addr_remote=3  link_addr_local=1  ip_addr_local='160.36.56.200'  tcp_port_local=18000  dnp3_options=0
  OpDNP3_AsyncSlaveCtrl1 : rtio_generic_dnp3/OpDNP3_AsyncSlaveCtrl  dev_id=5  nbr_aout=10  nbr_bout=1  cfg_name='AsyncDNP3_Slave_cfg.xml'  exe_name='AsyncDNP3_Slave'  nic_name='eth3'  link_addr_remote=11  link_addr_local=12  ip_addr_local='160.36.56.208'  tcp_port_local=18000  dnp3_options=0
  PV Farm 2 MW1 : Subsystem
      mask help: The product of the effeciency, the area covered by the Pv farm and the irradiance in w/m2 will give you the power generate by the PV farm
      mask DialogControl DescTextVar Prompt: The product of the efficiency, the area covered by the PV farm and the irradiance in W/m2 will give you the power generated by the PV farm.
      mask Display: image(imread('PV.jpg'))
  SSN Interface Block (3ph)1 : ssn_lib/SSN Interface Block (3ph)  nb_phase=3  nb_port=3  p1_type=V-type(Left)  p2_type=V-type (Right)  p3_type=V-type (Right)  p4_type=V-type(Left)  p5_type=V-type(Left)  p6_type=V-type(Left)  p7_type=V-type(Left)  p8_type=V-type(Left)  p9_type=V-type(Left)  p10_type=V-type(Left)  p11_type=V-type(Left)  p12_type=V-type(Left)  p13_type=V-type(Left)  p14_type=V-type(Left)  p15_type=V-type(Left)  p16_type=V-type(Left)  I_port_shunt_resistance=1e9
  SSN Interface Block (3ph){2..7} (6 alike) : ssn_lib/SSN Interface Block (3ph)  nb_phase=3  nb_port=2  p1_type=V-type(Left)  p2_type=V-type (Right)  p3_type=V-type(Left)  p4_type=V-type(Left)  p5_type=V-type(Left)  p6_type=V-type(Left)  p7_type=V-type(Left)  p8_type=V-type(Left)  p9_type=V-type(Left)  p10_type=V-type(Left)  p11_type=V-type(Left)  p12_type=V-type(Left)  p13_type=V-type(Left)  p14_type=V-type(Left)  p15_type=V-type(Left)  p16_type=V-type(Left)  I_port_shunt_resistance=1e9
  Step1 : Step  Commented=on  Time=0.5  SampleTime=0
  Step2 : Step  Time=9  Before=1  After=0  SampleTime=0
  Step3 : Step  SampleTime=0
  StubLine : artemis/ARTEMIS/StubLine  Commented=on  Phases=1  pu=off  L=1.2562*1806*ft2km/1.60934/Omega  Lpu=0.08  R=1.0582*1806*ft2km/1.60934  Rpu=0.002  S_base=450e6/3  V_base=230e3/sqrt(3)  F_base=60  Ts=1e-4
  StubLine1 : artemis/ARTEMIS/StubLine  Commented=on  Phases=1  pu=off  L=1.2562*2463*ft2km/1.60934/Omega  Lpu=0.08  R=1.0582*2463*ft2km/1.60934  Rpu=0.002  S_base=450e6/3  V_base=230e3/sqrt(3)  F_base=60  Ts=1e-4
  Substation : powerlib/Electrical Sources/Three-Phase Source  InternalConnection=Yg  VoltagePhases=on  Voltage=12.47e3  PhaseAngle=0  Voltage_phases=[ 1 1 1]*7200  PhaseAngles_phases=[ 0 -120 120]  Frequency=60  NonIdealSource=on  SpecifyImpedance=off  Resistance=2  Inductance=10/2/pi/60  ShortCircuitLevel=100e6  BaseVoltage=12.47e3  XRratio=7  BusType=swing  Pref=10e3  Qref=0  Prefabc=[3333.33 3333.33 3333.33]  Qrefabc=[0 0 0]  Qmin=-inf  Qmax=inf
  Subsystem : Subsystem
  Subsystem1 : Subsystem
  Subsystem2 : Subsystem
  Subsystem3 : Subsystem
  Subsystem4 : Subsystem
  Three-Phase Series RLC Branch : powerlib/Elements/Three-Phase Series RLC Branch  LConnTagsString=A|B|C  RConnTagsString=A|B|C  BranchType=RL  Resistance=R_OL(1)*220*ft2km  Inductance=X_OL(1)/Omega*220*ft2km  Capacitance=B_OL(1)/Omega*220*ft2km  Measurements=None
  Three-Phase Series RLC Branch1 : powerlib/Elements/Three-Phase Series RLC Branch  LConnTagsString=A|B|C  RConnTagsString=A|B|C  BranchType=RL  Resistance=R_OL(1)*174*ft2km  Inductance=X_OL(1)/Omega*174*ft2km  Capacitance=B_OL(1)/Omega*220*ft2km  Measurements=None
  Three-Phase Series RLC Branch10 : powerlib/Elements/Three-Phase Series RLC Branch  LConnTagsString=A|B|C  RConnTagsString=A|B|C  BranchType=RL  Resistance=R_OL(1)*591*ft2km  Inductance=X_OL(1)/Omega*591*ft2km  Capacitance=B_OL(1)/Omega*220*ft2km  Measurements=None
  Three-Phase Series RLC Branch11 : powerlib/Elements/Three-Phase Series RLC Branch  LConnTagsString=A|B|C  RConnTagsString=A|B|C  BranchType=RL  Resistance=R_OL(1)*664*ft2km  Inductance=X_OL(1)/Omega*664*ft2km  Capacitance=B_OL(1)/Omega*220*ft2km  Measurements=None
  Three-Phase Series RLC Branch12 : powerlib/Elements/Three-Phase Series RLC Branch  LConnTagsString=A|B|C  RConnTagsString=A|B|C  BranchType=RL  Resistance=R_OL(1)*172*ft2km  Inductance=X_OL(1)/Omega*172*ft2km  Capacitance=B_OL(1)/Omega*220*ft2km  Measurements=None
  Three-Phase Series RLC Branch13 : powerlib/Elements/Three-Phase Series RLC Branch  LConnTagsString=A|B|C  RConnTagsString=A|B|C  BranchType=RL  Resistance=R_OL(1)*2272*ft2km  Inductance=X_OL(1)/Omega*2272*ft2km  Capacitance=B_OL(1)/Omega*220*ft2km  Measurements=None
  Three-Phase Series RLC Branch14 : powerlib/Elements/Three-Phase Series RLC Branch  LConnTagsString=A|B|C  RConnTagsString=A|B|C  BranchType=RL  Resistance=R_OL(1)*197*ft2km  Inductance=X_OL(1)/Omega*197*ft2km  Capacitance=B_OL(1)/Omega*220*ft2km  Measurements=None
  Three-Phase Series RLC Branch15 : powerlib/Elements/Three-Phase Series RLC Branch  LConnTagsString=A|B|C  RConnTagsString=A|B|C  BranchType=RL  Resistance=R_OL(1)*272*ft2km  Inductance=X_OL(1)/Omega*272*ft2km  Capacitance=B_OL(1)/Omega*220*ft2km  Measurements=None
  Three-Phase Series RLC Branch16 : powerlib/Elements/Three-Phase Series RLC Branch  LConnTagsString=A|B|C  RConnTagsString=A|B|C  BranchType=RL  Resistance=R/150  Inductance=5.4568e-05/2  Capacitance=1e-6  Measurements=None
  Three-Phase Series RLC Branch17 : powerlib/Elements/Three-Phase Series RLC Branch  LConnTagsString=A|B|C  RConnTagsString=A|B|C  BranchType=RL  Resistance=R/150  Inductance=5.4568e-05/2  Capacitance=1e-6  Measurements=None
  Three-Phase Series RLC Branch18 : powerlib/Elements/Three-Phase Series RLC Branch  LConnTagsString=A|B|C  RConnTagsString=A|B|C  BranchType=RL  Resistance=R*30  Inductance=L*30  Capacitance=1e-6  Measurements=None
  Three-Phase Series RLC Branch19 : powerlib/Elements/Three-Phase Series RLC Branch  LConnTagsString=A|B|C  RConnTagsString=A|B|C  BranchType=RL  Resistance=R_OL(1)*1943*ft2km  Inductance=X_OL(1)/Omega*1943*ft2km  Capacitance=B_OL(1)/Omega*220*ft2km  Measurements=None
  Three-Phase Series RLC Branch2 : powerlib/Elements/Three-Phase Series RLC Branch  LConnTagsString=A|B|C  RConnTagsString=A|B|C  BranchType=RL  Resistance=R_OL(1)*920*ft2km  Inductance=X_OL(1)/Omega*920*ft2km  Capacitance=B_OL(1)/Omega*220*ft2km  Measurements=None
  Three-Phase Series RLC Branch20 : powerlib/Elements/Three-Phase Series RLC Branch  LConnTagsString=A|B|C  RConnTagsString=A|B|C  BranchType=RL  Resistance=R_OL(1)*1211*ft2km  Inductance=X_OL(1)/Omega*1211*ft2km  Capacitance=B_OL(1)/Omega*220*ft2km  Measurements=None
  Three-Phase Series RLC Branch21 : powerlib/Elements/Three-Phase Series RLC Branch  LConnTagsString=A|B|C  RConnTagsString=A|B|C  BranchType=RL  Resistance=R_OL(1)*483*ft2km  Inductance=X_OL(1)/Omega*483*ft2km  Capacitance=B_OL(1)/Omega*220*ft2km  Measurements=None
  Three-Phase Series RLC Branch22 : powerlib/Elements/Three-Phase Series RLC Branch  LConnTagsString=A|B|C  RConnTagsString=A|B|C  BranchType=RL  Resistance=R_OL(1)*1274*ft2km  Inductance=X_OL(1)/Omega*1274*ft2km  Capacitance=B_OL(1)/Omega*220*ft2km  Measurements=None
  Three-Phase Series RLC Branch23 : powerlib/Elements/Three-Phase Series RLC Branch  LConnTagsString=A|B|C  RConnTagsString=A|B|C  BranchType=RL  Resistance=R_OL(1)*1932*ft2km  Inductance=X_OL(1)/Omega*1932*ft2km  Capacitance=B_OL(1)/Omega*220*ft2km  Measurements=None
  Three-Phase Series RLC Branch24 : powerlib/Elements/Three-Phase Series RLC Branch  LConnTagsString=A|B|C  RConnTagsString=A|B|C  BranchType=RL  Resistance=R_OL(1)*668*ft2km  Inductance=X_OL(1)/Omega*668*ft2km  Capacitance=B_OL(1)/Omega*220*ft2km  Measurements=None
  Three-Phase Series RLC Branch25 : powerlib/Elements/Three-Phase Series RLC Branch  LConnTagsString=A|B|C  RConnTagsString=A|B|C  BranchType=RL  Resistance=R_OL(1)*997*ft2km  Inductance=X_OL(1)/Omega*997*ft2km  Capacitance=B_OL(1)/Omega*220*ft2km  Measurements=None
  Three-Phase Series RLC Branch26 : powerlib/Elements/Three-Phase Series RLC Branch  LConnTagsString=A|B|C  RConnTagsString=A|B|C  BranchType=RL  Resistance=R_OL(1)*308*ft2km  Inductance=X_OL(1)/Omega*308*ft2km  Capacitance=B_OL(1)/Omega*220*ft2km  Measurements=None
  Three-Phase Series RLC Branch27 : powerlib/Elements/Three-Phase Series RLC Branch  LConnTagsString=A|B|C  RConnTagsString=A|B|C  BranchType=RL  Resistance=R_OL(1)*359*ft2km  Inductance=X_OL(1)/Omega*359*ft2km  Capacitance=B_OL(1)/Omega*220*ft2km  Measurements=None
  Three-Phase Series RLC Branch28 : powerlib/Elements/Three-Phase Series RLC Branch  LConnTagsString=A|B|C  RConnTagsString=A|B|C  BranchType=RL  Resistance=R_OL(1)*702*ft2km  Inductance=X_OL(1)/Omega*702*ft2km  Capacitance=B_OL(1)/Omega*220*ft2km  Measurements=None
  Three-Phase Series RLC Branch29 : powerlib/Elements/Three-Phase Series RLC Branch  LConnTagsString=A|B|C  RConnTagsString=A|B|C  BranchType=RL  Resistance=R_OL(1)*622*ft2km  Inductance=X_OL(1)/Omega*622*ft2km  Capacitance=B_OL(1)/Omega*220*ft2km  Measurements=None
  Three-Phase Series RLC Branch3 : powerlib/Elements/Three-Phase Series RLC Branch  LConnTagsString=A|B|C  RConnTagsString=A|B|C  BranchType=RL  Resistance=R_OL(1)*2257*ft2km  Inductance=X_OL(1)/Omega*2257*ft2km  Capacitance=B_OL(1)/Omega*220*ft2km  Measurements=None
  Three-Phase Series RLC Branch30 : powerlib/Elements/Three-Phase Series RLC Branch  LConnTagsString=A|B|C  RConnTagsString=A|B|C  BranchType=RL  Resistance=R_OL(1)*630*ft2km  Inductance=X_OL(1)/Omega*630*ft2km  Capacitance=B_OL(1)/Omega*220*ft2km  Measurements=None
  Three-Phase Series RLC Branch4 : powerlib/Elements/Three-Phase Series RLC Branch  LConnTagsString=A|B|C  RConnTagsString=A|B|C  BranchType=RL  Resistance=R_OL(1)*172*ft2km  Inductance=X_OL(1)/Omega*172*ft2km  Capacitance=B_OL(1)/Omega*220*ft2km  Measurements=None
  Three-Phase Series RLC Branch5 : powerlib/Elements/Three-Phase Series RLC Branch  LConnTagsString=A|B|C  RConnTagsString=A|B|C  BranchType=RL  Resistance=R_OL(1)*882*ft2km  Inductance=X_OL(1)/Omega*882*ft2km  Capacitance=B_OL(1)/Omega*220*ft2km  Measurements=None
  Three-Phase Series RLC Branch6 : powerlib/Elements/Three-Phase Series RLC Branch  LConnTagsString=A|B|C  RConnTagsString=A|B|C  BranchType=RL  Resistance=R_OL(1)*249*ft2km  Inductance=X_OL(1)/Omega*249*ft2km  Capacitance=B_OL(1)/Omega*220*ft2km  Measurements=None
  Three-Phase Series RLC Branch9 : powerlib/Elements/Three-Phase Series RLC Branch  LConnTagsString=A|B|C  RConnTagsString=A|B|C  BranchType=RL  Resistance=R_OL(1)*1000*ft2km  Inductance=X_OL(1)/Omega*1000*ft2km  Capacitance=B_OL(1)/Omega*220*ft2km  Measurements=None
  Three-Phase Transformer (Two Windings) : powerlib/Elements/Three-Phase Transformer (Two Windings)  Winding1Connection=Yg  Winding2Connection=Yg  CoreType=Three single-phase transformers  SetSaturation=off  Hysteresis=off  DataFile='hysteresis'  SetInitialFlux=off  Measurements=None  UNITS=pu  NominalPower=[ 600e3 , 60 ]  Winding1=[ 12.47e3 , 0.002 , 0.01 ]  Winding2=[ 480 , 0.002 , 0.01 ]  Rm=500  Lm=500  L0=0.5  Saturation=[ 0,0 ; 0.0024,1.2 ; 1.0,1.52 ]  InitialFluxes=[ 0.8 , -0.8 , 0.7 ]  MoreParameters=off  BreakLoop=off  DataType=off  TransfoNumber=1
  Three-Phase Transformer (Two Windings)2 : powerlib/Elements/Three-Phase Transformer (Two Windings)  Winding1Connection=Yg  Winding2Connection=Yg  CoreType=Three single-phase transformers  SetSaturation=off  Hysteresis=off  DataFile='hysteresis'  SetInitialFlux=off  Measurements=None  UNITS=pu  NominalPower=[ 600e3 , 60 ]  Winding1=[ 12.47e3 , 0.002 , 0.01 ]  Winding2=[ 480 , 0.002 , 0.01 ]  Rm=500  Lm=500  L0=0.5  Saturation=[ 0,0 ; 0.0024,1.2 ; 1.0,1.52 ]  InitialFluxes=[ 0.8 , -0.8 , 0.7 ]  MoreParameters=off  BreakLoop=off  DataType=off  TransfoNumber=1
  Three-Phase Transformer (Two Windings)3 : powerlib/Elements/Three-Phase Transformer (Two Windings)  Winding1Connection=Delta (D1)  Winding2Connection=Yg  CoreType=Three single-phase transformers  SetSaturation=off  Hysteresis=off  DataFile='hysteresis'  SetInitialFlux=on  Measurements=None  UNITS=pu  NominalPower=[ 300e3 , 60 ]  Winding1=[12200 0.00087718*2.6 0.0029794*2.6]  Winding2=[12200 0.0026316*2.6 0.0089382*2.6]  Rm=500  Lm=500.01  L0=0.50001  Saturation=[0 0;1.1467e-08 5.9765e-09;4.7776e-06 7.5711e-09]  InitialFluxes=[-0.018019 0.019537 -0.0015725]  MoreParameters=off  BreakLoop=off  DataType=off  TransfoNumber=1
  Three-Phase Transformer (Two Windings)4 : powerlib/Elements/Three-Phase Transformer (Two Windings)  Winding1Connection=Delta (D1)  Winding2Connection=Yg  CoreType=Three single-phase transformers  SetSaturation=off  Hysteresis=off  DataFile='hysteresis'  SetInitialFlux=on  Measurements=None  UNITS=pu  NominalPower=[ 300e3 , 60 ]  Winding1=[12200 0.00087718*2.6 0.0029794*2.6]  Winding2=[12200 0.0026316*2.6 0.0089382*2.6]  Rm=500  Lm=500.01  L0=0.50001  Saturation=[0 0;1.1467e-08 5.9765e-09;4.7776e-06 7.5711e-09]  InitialFluxes=[-0.018019 0.019537 -0.0015725]  MoreParameters=off  BreakLoop=off  DataType=off  TransfoNumber=1
  Three-Phase Fault3 : powerlib/Elements/Three-Phase Fault  Commented=on  InitialStates=0  FaultA=on  FaultB=on  FaultC=on  GroundFault=on  SwitchTimes="[1/60  5/60]"  External=on  SwitchStatus=NaN  FaultResistance=0.001  GroundResistance=0.01  SnubberResistance=1e6  SnubberCapacitance=inf  Measurements=None
  Triplex 10 : powerlib/Elements/Three-Phase Series RLC Load  LConnTagsString=A|B|C  Configuration=Y (grounded)  NominalVoltage=480  Vabc=[1 1 1]*120  Vabcp=[1e3 1e3 1e3]  NominalFrequency=60  UnbalancedPower=on  ActivePower=10e3  InductivePower=100  CapacitivePower=100  Pabc=[33716.4993 41582.0851 34666.3646]*load_scale/2  QLabc=[21799.9726 26952.4912 22381.7649]*load_scale/10  QCabc=[0 0 0]  Pabcp=[10e3 9e3 11e3]  QLabcp=[100 90 110]  QCabcp=[100 90 110]  Measurements=None  LoadType=constant Z
  Triplex 11 : powerlib/Elements/Three-Phase Series RLC Load  LConnTagsString=A|B|C  Configuration=Y (grounded)  NominalVoltage=480  Vabc=[1 1 1]*120  Vabcp=[1e3 1e3 1e3]  NominalFrequency=60  UnbalancedPower=on  ActivePower=10e3  InductivePower=100  CapacitivePower=100  Pabc=[99203.4648 122346.2398 101998.2367]*load_scale  QLabc=[64141.677 79301.8422 65853.4744]*load_scale/10  QCabc=[0 0 0]  Pabcp=[10e3 9e3 11e3]  QLabcp=[100 90 110]  QCabcp=[100 90 110]  Measurements=None  LoadType=constant Z
  Triplex 12 : powerlib/Elements/Three-Phase Series RLC Load  LConnTagsString=A|B|C  Configuration=Y (grounded)  NominalVoltage=480  Vabc=[1 1 1]*120  Vabcp=[1e3 1e3 1e3]  NominalFrequency=60  UnbalancedPower=on  ActivePower=10e3  InductivePower=100  CapacitivePower=100  Pabc=[90321.0027 111391.624 92865.5368]*load_scale  QLabc=[58398.571 72201.328 59957.0978]*load_scale/10  QCabc=[0 0 0]  Pabcp=[10e3 9e3 11e3]  QLabcp=[100 90 110]  QCabcp=[100 90 110]  Measurements=None  LoadType=constant Z
  Triplex 13 : powerlib/Elements/Three-Phase Series RLC Load  LConnTagsString=A|B|C  Configuration=Y (grounded)  NominalVoltage=480  Vabc=[1 1 1]*120  Vabcp=[1e3 1e3 1e3]  NominalFrequency=60  UnbalancedPower=on  ActivePower=10e3  InductivePower=100  CapacitivePower=100  Pabc=[17447.9567 21518.3199 17939.5026]*load_scale  QLabc=[11281.2713 13947.649 11582.3431]*load_scale/10  QCabc=[0 0 0]  Pabcp=[10e3 9e3 11e3]  QLabcp=[100 90 110]  QCabcp=[100 90 110]  Measurements=None  LoadType=constant Z
  Triplex 14 : powerlib/Elements/Three-Phase Series RLC Load  LConnTagsString=A|B|C  Configuration=Y (grounded)  NominalVoltage=480  Vabc=[1 1 1]*120  Vabcp=[1e3 1e3 1e3]  NominalFrequency=60  UnbalancedPower=on  ActivePower=10e3  InductivePower=100  CapacitivePower=100  Pabc=[83871.0821 103437.0275 86233.9082]*load_scale  QLabc=[54228.2658 67045.353 55675.4965]*load_scale/10  QCabc=[0 0 0]  Pabcp=[10e3 9e3 11e3]  QLabcp=[100 90 110]  QCabcp=[100 90 110]  Measurements=None  LoadType=constant Z
  Triplex 2 : powerlib/Elements/Series RLC Load  Commented=on  LConnTagsString=a  RConnTagsString=__new0  NominalVoltage=120  NominalFrequency=60  ActivePower=3157.18*load_scale  InductivePower=2041.33*load_scale/10  CapacitivePower=0  Setx0=off  InitialVoltage=0  SetiL0=off  InitialCurrent=0  Measurements=None  LoadType=constant Z
  Triplex 3 : powerlib/Elements/Series RLC Load  Commented=on  LConnTagsString=a  RConnTagsString=__new0  NominalVoltage=120  NominalFrequency=60  ActivePower=5020.58*load_scale  InductivePower=2907.27*load_scale/10  CapacitivePower=0  Setx0=off  InitialVoltage=0  SetiL0=off  InitialCurrent=0  Measurements=None  LoadType=constant Z
  Triplex 4 : powerlib/Elements/Series RLC Load  Commented=on  LConnTagsString=a  RConnTagsString=__new0  NominalVoltage=120  NominalFrequency=60  ActivePower=2273.32*load_scale  InductivePower=1502.1*load_scale/10  CapacitivePower=0  Setx0=off  InitialVoltage=0  SetiL0=off  InitialCurrent=0  Measurements=None  LoadType=constant Z
  Triplex 5 : powerlib/Elements/Series RLC Load  Commented=on  LConnTagsString=a  RConnTagsString=__new0  NominalVoltage=120  NominalFrequency=60  ActivePower=4976.67*load_scale  InductivePower=3213.1*load_scale/10  CapacitivePower=0  Setx0=off  InitialVoltage=0  SetiL0=off  InitialCurrent=0  Measurements=None  LoadType=constant Z
  Triplex 6 : powerlib/Elements/Three-Phase Series RLC Load  LConnTagsString=A|B|C  Configuration=Y (grounded)  NominalVoltage=480  Vabc=[1 1 1]*120  Vabcp=[1e3 1e3 1e3]  NominalFrequency=60  UnbalancedPower=on  ActivePower=10e3  InductivePower=100  CapacitivePower=100  Pabc=[139237.2007 171719.284 143159.8077]*load_scale/2  QLabc=[90026.1657 111304.2427 92428.762]*load_scale/10  QCabc=[0 0 0]  Pabcp=[10e3 9e3 11e3]  QLabcp=[100 90 110]  QCabcp=[100 90 110]  Measurements=None  LoadType=constant Z
  Triplex 7 : powerlib/Elements/Three-Phase Series RLC Load  LConnTagsString=A|B|C  Configuration=Y (grounded)  NominalVoltage=480  Vabc=[1 1 1]*120  Vabcp=[1e3 1e3 1e3]  NominalFrequency=60  UnbalancedPower=on  ActivePower=10e3  InductivePower=100  CapacitivePower=100  Pabc=[55911.5976 68954.988 57486.7458]*load_scale/2  QLabc=[36150.5885 44694.9378 37115.3666]*load_scale/10  QCabc=[0 0 0]  Pabcp=[10e3 9e3 11e3]  QLabcp=[100 90 110]  QCabcp=[100 90 110]  Measurements=None  LoadType=constant Z
  Triplex 8 : powerlib/Elements/Three-Phase Series RLC Load  LConnTagsString=A|B|C  Configuration=Y (grounded)  NominalVoltage=480  Vabc=[1 1 1]*120  Vabcp=[1e3 1e3 1e3]  NominalFrequency=60  UnbalancedPower=on  ActivePower=10e3  InductivePower=100  CapacitivePower=100  Pabc=[43896.3169 54136.7111 45132.9692]*load_scale/2  QLabc=[28381.9057 35090.0929 29139.3551]*load_scale/10  QCabc=[0 0 0]  Pabcp=[10e3 9e3 11e3]  QLabcp=[100 90 110]  QCabcp=[100 90 110]  Measurements=None  LoadType=constant Z
  Triplex 9 : powerlib/Elements/Three-Phase Series RLC Load  LConnTagsString=A|B|C  Configuration=Y (grounded)  NominalVoltage=480  Vabc=[1 1 1]*120  Vabcp=[1e3 1e3 1e3]  NominalFrequency=60  UnbalancedPower=on  ActivePower=10e3  InductivePower=100  CapacitivePower=100  Pabc=[50051.384 61727.6689 51461.4376]*load_scale/2  QLabc=[32361.5684 40010.3662 33225.226]*load_scale/10  QCabc=[0 0 0]  Pabcp=[10e3 9e3 11e3]  QLabcp=[100 90 110]  QCabcp=[100 90 110]  Measurements=None  LoadType=constant Z
  V1 : powerlib/Electrical Sources/Controlled Voltage Source  Initialize=on  Source_Type=AC  Amplitude=0  Phase=0  Frequency=0  Measurements=None
  V2 : powerlib/Electrical Sources/Controlled Voltage Source  Initialize=on  Source_Type=AC  Amplitude=0  Phase=0  Frequency=0  Measurements=None
  V3 : powerlib/Electrical Sources/Controlled Voltage Source  Initialize=on  Source_Type=AC  Amplitude=0  Phase=0  Frequency=0  Measurements=None
  VI_BESS2 : powerlib/Measurements/Three-Phase V-I Measurement  VoltageMeasurement=phase-to-ground  SetLabelV=on  LabelV=Vabc_BESS2  Vpu=off  VpuLL=off  CurrentMeasurement=yes  SetLabelI=on  LabelI=Iabc_BESS2  Ipu=off  Pbase=100e6  Vbase=Vabc_B  OutputType=Complex  PhasorSimulation=off  PSBequivalent=0
  VI_BESS4 : powerlib/Measurements/Three-Phase V-I Measurement  VoltageMeasurement=phase-to-ground  SetLabelV=on  LabelV=Vabc_BESS3_sec1  Vpu=off  VpuLL=off  CurrentMeasurement=yes  SetLabelI=on  LabelI=Iabc_BESS3_sec1  Ipu=off  Pbase=100e6  Vbase=480  OutputType=Complex  PhasorSimulation=off  PSBequivalent=0
  VI_BESS6 : powerlib/Measurements/Three-Phase V-I Measurement  VoltageMeasurement=phase-to-ground  SetLabelV=on  LabelV=Vabc_BESS3_sec  Vpu=off  VpuLL=off  CurrentMeasurement=yes  SetLabelI=on  LabelI=Iabc_BESS3_sec  Ipu=off  Pbase=100e6  Vbase=480  OutputType=Complex  PhasorSimulation=off  PSBequivalent=0
  VI_PV1 : powerlib/Measurements/Three-Phase V-I Measurement  VoltageMeasurement=phase-to-phase  SetLabelV=on  LabelV=Vabc_PV1  Vpu=on  VpuLL=off  CurrentMeasurement=yes  SetLabelI=on  LabelI=Iabc_PV1  Ipu=off  Pbase=100e6  Vbase=Vabc_B  OutputType=Complex  PhasorSimulation=off  PSBequivalent=0
  VI_Y1L1 : powerlib/Measurements/Three-Phase V-I Measurement  VoltageMeasurement=phase-to-ground  SetLabelV=on  LabelV=Vabc_Y1_L  Vpu=on  VpuLL=off  CurrentMeasurement=yes  SetLabelI=on  LabelI=Iabc_Y1_L  Ipu=off  Pbase=100e6  Vbase=Vabc_B  OutputType=Complex  PhasorSimulation=off  PSBequivalent=0
  VI_Y1R1 : powerlib/Measurements/Three-Phase V-I Measurement  VoltageMeasurement=phase-to-ground  SetLabelV=on  LabelV=Vabc_Y1_R  Vpu=on  VpuLL=off  CurrentMeasurement=yes  SetLabelI=on  LabelI=Iabc_Y1_R  Ipu=off  Pbase=100e6  Vbase=Vabc_B  OutputType=Complex  PhasorSimulation=off  PSBequivalent=0
  VI_Y2L1 : powerlib/Measurements/Three-Phase V-I Measurement  VoltageMeasurement=phase-to-ground  SetLabelV=on  LabelV=Vabc_Y2_L  Vpu=on  VpuLL=off  CurrentMeasurement=yes  SetLabelI=on  LabelI=Iabc_Y2_L  Ipu=off  Pbase=100e6  Vbase=Vabc_B  OutputType=Complex  PhasorSimulation=off  PSBequivalent=0
  VI_Y2R1 : powerlib/Measurements/Three-Phase V-I Measurement  VoltageMeasurement=phase-to-ground  SetLabelV=on  LabelV=Vabc_Y2_R  Vpu=on  VpuLL=off  CurrentMeasurement=yes  SetLabelI=on  LabelI=Iabc_Y2_R  Ipu=off  Pbase=100e6  Vbase=Vabc_B  OutputType=Complex  PhasorSimulation=off  PSBequivalent=0
  VI_Y3L1 : powerlib/Measurements/Three-Phase V-I Measurement  VoltageMeasurement=phase-to-ground  SetLabelV=on  LabelV=Vabc_Y3_L  Vpu=on  VpuLL=off  CurrentMeasurement=yes  SetLabelI=on  LabelI=Iabc_Y3_L  Ipu=off  Pbase=100e6  Vbase=Vabc_B  OutputType=Complex  PhasorSimulation=off  PSBequivalent=0
  VI_Y3R1 : powerlib/Measurements/Three-Phase V-I Measurement  VoltageMeasurement=phase-to-ground  SetLabelV=on  LabelV=Vabc_Y3_R  Vpu=on  VpuLL=off  CurrentMeasurement=yes  SetLabelI=on  LabelI=Iabc_Y3_R  Ipu=off  Pbase=100e6  Vbase=Vabc_B  OutputType=Complex  PhasorSimulation=off  PSBequivalent=0
  VI_Y4L : powerlib/Measurements/Three-Phase V-I Measurement  VoltageMeasurement=phase-to-ground  SetLabelV=on  LabelV=Vabc_Y4_L  Vpu=on  VpuLL=off  CurrentMeasurement=yes  SetLabelI=on  LabelI=Iabc_Y4_L  Ipu=off  Pbase=100e6  Vbase=Vabc_B  OutputType=Complex  PhasorSimulation=off  PSBequivalent=0
  VI_Y4R : powerlib/Measurements/Three-Phase V-I Measurement  VoltageMeasurement=phase-to-ground  SetLabelV=on  LabelV=Vabc_Y4_R  Vpu=on  VpuLL=off  CurrentMeasurement=yes  SetLabelI=on  LabelI=Iabc_Y4_R  Ipu=off  Pbase=100e6  Vbase=Vabc_B  OutputType=Complex  PhasorSimulation=off  PSBequivalent=0
  VI_Y4R1 : powerlib/Measurements/Three-Phase V-I Measurement  VoltageMeasurement=phase-to-ground  SetLabelV=on  LabelV=Vabc_Y4_R1  Vpu=on  VpuLL=off  CurrentMeasurement=yes  SetLabelI=on  LabelI=Iabc_Y4_R1  Ipu=off  Pbase=100e6  Vbase=Vabc_B  OutputType=Complex  PhasorSimulation=off  PSBequivalent=0
  VI_Y4R2 : powerlib/Measurements/Three-Phase V-I Measurement  VoltageMeasurement=phase-to-ground  SetLabelV=on  LabelV=Vabc_Y4_R2  Vpu=on  VpuLL=off  CurrentMeasurement=yes  SetLabelI=on  LabelI=Iabc_Y4_R2  Ipu=off  Pbase=100e6  Vbase=Vabc_B  OutputType=Complex  PhasorSimulation=off  PSBequivalent=0
  VI_Y5L : powerlib/Measurements/Three-Phase V-I Measurement  VoltageMeasurement=phase-to-ground  SetLabelV=on  LabelV=Vabc_Y5_L  Vpu=on  VpuLL=off  CurrentMeasurement=yes  SetLabelI=on  LabelI=Iabc_Y5_L  Ipu=off  Pbase=100e6  Vbase=Vabc_B  OutputType=Complex  PhasorSimulation=off  PSBequivalent=0
  VI_Y5R : powerlib/Measurements/Three-Phase V-I Measurement  VoltageMeasurement=phase-to-ground  SetLabelV=on  LabelV=Vabc_Y5_R  Vpu=on  VpuLL=off  CurrentMeasurement=yes  SetLabelI=on  LabelI=Iabc_Y5_R  Ipu=off  Pbase=100e6  Vbase=Vabc_B  OutputType=Complex  PhasorSimulation=off  PSBequivalent=0
  VI_Y6L : powerlib/Measurements/Three-Phase V-I Measurement  VoltageMeasurement=phase-to-ground  SetLabelV=on  LabelV=Vabc_Y6_L  Vpu=on  VpuLL=off  CurrentMeasurement=yes  SetLabelI=on  LabelI=Iabc_Y6_L  Ipu=off  Pbase=100e6  Vbase=Vabc_B  OutputType=Complex  PhasorSimulation=off  PSBequivalent=0
  VI_Y6R : powerlib/Measurements/Three-Phase V-I Measurement  VoltageMeasurement=phase-to-ground  SetLabelV=on  LabelV=Vabc_Y6_R  Vpu=on  VpuLL=off  CurrentMeasurement=yes  SetLabelI=on  LabelI=Iabc_Y6_R  Ipu=off  Pbase=100e6  Vbase=Vabc_B  OutputType=Complex  PhasorSimulation=off  PSBequivalent=0
  VI_Y7L1 : powerlib/Measurements/Three-Phase V-I Measurement  VoltageMeasurement=phase-to-ground  SetLabelV=on  LabelV=Vabc_Y7_L  Vpu=on  VpuLL=off  CurrentMeasurement=yes  SetLabelI=on  LabelI=Iabc_Y7_L  Ipu=off  Pbase=100e6  Vbase=Vabc_B  OutputType=Complex  PhasorSimulation=off  PSBequivalent=0
  VI_Y7R1 : powerlib/Measurements/Three-Phase V-I Measurement  VoltageMeasurement=phase-to-ground  SetLabelV=on  LabelV=Vabc_Y7_R  Vpu=on  VpuLL=off  CurrentMeasurement=yes  SetLabelI=on  LabelI=Iabc_Y7_R  Ipu=off  Pbase=100e6  Vbase=Vabc_B  OutputType=Complex  PhasorSimulation=off  PSBequivalent=0
  VI_Y8L : powerlib/Measurements/Three-Phase V-I Measurement  VoltageMeasurement=phase-to-ground  SetLabelV=on  LabelV=Vabc_Y8_L  Vpu=on  VpuLL=off  CurrentMeasurement=yes  SetLabelI=on  LabelI=Iabc_Y8_L  Ipu=off  Pbase=100e6  Vbase=Vabc_B  OutputType=Complex  PhasorSimulation=off  PSBequivalent=0
  VI_Y8R : powerlib/Measurements/Three-Phase V-I Measurement  VoltageMeasurement=phase-to-ground  SetLabelV=on  LabelV=Vabc_Y8_R  Vpu=on  VpuLL=off  CurrentMeasurement=yes  SetLabelI=on  LabelI=Iabc_Y8_R  Ipu=off  Pbase=100e6  Vbase=Vabc_B  OutputType=Complex  PhasorSimulation=off  PSBequivalent=0
  Voltage and Current Bus1 : Scope  NumInputPorts=3
  Voltage and Current Bus4 : Scope  NumInputPorts=3
  Y{1,6,12,21} (4 alike) : powerlib/Elements/Three-Phase Breaker  InitialState=closed  SwitchA=on  SwitchB=on  SwitchC=on  SwitchTimes=0.5  External=on  BreakerResistance=0.00001  SnubberResistance=1e6  SnubberCapacitance=inf  Measurements=None
  Y{2..3,10,22..25} (7 alike) : powerlib/Elements/Three-Phase Breaker  InitialState=closed  SwitchA=on  SwitchB=on  SwitchC=on  SwitchTimes=10  External=on  BreakerResistance=0.00001  SnubberResistance=1e6  SnubberCapacitance=inf  Measurements=None
  Y16 : powerlib/Elements/Three-Phase Breaker  InitialState=open  SwitchA=on  SwitchB=on  SwitchC=on  SwitchTimes=10  External=on  BreakerResistance=0.00001  SnubberResistance=1e6  SnubberCapacitance=inf  Measurements=None
  Y20 : powerlib/Elements/Three-Phase Breaker  InitialState=open  SwitchA=on  SwitchB=on  SwitchC=on  SwitchTimes=10  External=on  BreakerResistance=1e-6  SnubberResistance=1e6  SnubberCapacitance=inf  Measurements=None
  Y4 : powerlib/Elements/Three-Phase Breaker  InitialState=open  SwitchA=on  SwitchB=on  SwitchC=on  SwitchTimes=10  External=on  BreakerResistance=1e-6  SnubberResistance=1e6  SnubberCapacitance=inf  Measurements=None
  Y5 : powerlib/Elements/Three-Phase Breaker  InitialState=open  SwitchA=on  SwitchB=on  SwitchC=on  SwitchTimes=10  External=on  BreakerResistance=0.00001  SnubberResistance=1e6  SnubberCapacitance=inf  Measurements=None
  SM2SC : Outport
  SM2SS : Outport  Port=2
  tag scope: Angle_diff=global, Comm_SW_Out=global, F3=global, F5=global, F6=global, F7=global, Freq_diff=global, G1_En=global, Gen_F=global, Gen_P=global, Gen_V=global, Grid_enable=global, MG1_ISD=global, MG2_ISD=global, Manual_Reset=global, S_BESS1=global, S_BESS2=global, S_G1=global, S_G2=global, S_PV=global, S_Y1=global, S_Y2=global, S_Y3=global, S_Y4=global, S_Y5=global, S_Y6=global, S_Y7=global, S_Y8=global, V_BESS1=global, V_BESS2=global, V_mag_diff=global, V_mag_limit=global, Vref_PV1=global
  wires:
  SC2SM/1 -> OpComm1/1
  [Vabc_BESS3_sec] -> Voltage and Current Bus1/2, Mux1/1
  SS2SM/1 -> OpComm2/1
  [Iabc_BESS3_sec] -> Gain5/1
  OpComm2/1 -> Demux2/1
  Demux2/1 -> [S_BESS1]
  Demux2/2 -> [V_BESS1]
  OpComm1/1 -> Demux3/1
  [V_BESS2] -> Voltage and Current Bus1/1
  Gain5/1 -> Mux1/2, Voltage and Current Bus1/3
  Mux1/1 -> Memory/1
  Memory/1 -> SM2SS/1
  [Iabc_Y3_R] -> Mux2/1
  Memory1/1 -> SM2SC/1
  Demux2/3 -> [S_PV]
  Demux2/4 -> [Vref_PV1]
  [Iabc_PV1] -> Mux1/5
  [Vabc_PV1] -> Mux1/4
  Demux2/5 -> [S_BESS2]
  Demux2/6 -> [V_BESS2]
  [Vabc_BESS3_sec1] -> Mux1/6
  [Iabc_BESS3_sec1] -> Gain3/1
  Gain3/1 -> Mux1/7
  Data Type Conversion1/1 -> Mux1/8
  [S_BESS1] -> Mux1/9
  [S_BESS2] -> Mux1/10
  [S_BESS1] -> Y4/1
  [S_BESS2] -> Y20/1
  [S_Gen1] -> Y5/1
  [SW_Y2] -> Y22/1
  [SW_Y3] -> Y23/1
  [SW_Y4] -> Y24/1
  [SW_Y5] -> Y25/1
  [SW_Y6] -> Y10/1
  [S_PV] -> Y16/1
  [SW_Y7] -> Y12/1
  [SW_Y1] -> Y21/1
  Constant7/1 -> [V_mag_limit]
  Constant8/1 -> [V_mag_diff]
  Constant9/1 -> [Freq_diff]
  Constant10/1 -> [Angle_diff]
  Logical Operator8/1 -> Data Type Conversion1/1
  [SW_Y3] -> Logical Operator8/1
  [SW_Y1] -> Logical Operator8/2
  [SW_Y7] -> Logical Operator1/1
  [SW_Y1] -> Logical Operator1/2
  [S_PV] -> Mux1/11
  [Iabc_Y4_L] -> Voltage and Current Bus4/2
  [Vabc_Y4_L] -> Voltage and Current Bus4/1
  [S_G1] -> Y1/1
  [S_G2] -> Y2/1
  [SW_Y8] -> Y3/1
  Generator2/1(Vabc) -> Demux/1
  Demux/1 -> V1/1
  Demux/2 -> V2/1
  Demux/3 -> V3/1
  Logical Operator1/1 -> Data Type Conversion/1
  [SW_Y8] -> Logical Operator1/3
  [Iabc_Y8_L] -> Mux2/2
  [Iabc_Y1_L] -> Mux2/5
  [Iabc_Y5_R] -> Mux2/4
  [Y1s] -> Mux2/3
  [F3] -> Subsystem4/1(In1)
  [F5] -> Subsystem3/1(In1)
  [F7] -> Subsystem/1(In1)
  [F4] -> Subsystem1/1(In1)
  [F6] -> Subsystem2/1(In1)
  Demux2/7 -> Demux17/1
  Demux17/1 -> Logical Operator/1
  [Grid_enable] -> Y6/1
  Logical Operator/1 -> [MG1_ISD]
  Demux17/2 -> Logical Operator2/1
  Logical Operator2/1 -> [MG2_ISD]
  Analog outputs init values1/1 -> OpDNP3_AsyncSlaveCtrl/2, OpDNP3_AsyncSlaveCtrl/4
  Mux3/1 -> OpDNP3_AsyncSlaveCtrl/1
  OpDNP3_AsyncSlaveCtrl/2 -> Demux13/1, [Comm_SW_Out]
  Analog outputs init values2/1 -> OpDNP3_AsyncSlaveCtrl/3
  [m_Y1] -> Mux3/1
  [m_Y2] -> Mux3/2
  [m_Y3] -> Mux3/3
  [m_Y4] -> Mux3/4
  [m_Y5] -> Mux3/5
  [m_Y6] -> Mux3/6
  [m_Y7] -> Mux3/7
  [m_Y8] -> Mux3/8
  Demux13/10 -> Data Type Conversion10/1
  Demux13/1 -> Data Type Conversion3/1
  Demux13/2 -> Data Type Conversion4/1
  Demux13/3 -> Data Type Conversion5/1
  Demux13/4 -> Data Type Conversion6/1
  Demux13/5 -> Data Type Conversion7/1
  Demux13/6 -> Data Type Conversion8/1
  Demux13/7 -> Data Type Conversion9/1
  Demux13/8 -> Data Type Conversion11/1
  Demux13/9 -> Data Type Conversion12/1
  OpDNP3_AsyncSlaveCtrl/3 -> Data Type Conversion2/1
  Data Type Conversion2/1 -> ?
  Data Type Conversion3/1 -> [S_Y1]
  Data Type Conversion4/1 -> [S_Y2]
  Data Type Conversion5/1 -> [S_Y3]
  Data Type Conversion6/1 -> [S_Y4]
  Data Type Conversion7/1 -> [S_Y5]
  Data Type Conversion8/1 -> [S_Y6]
  Data Type Conversion9/1 -> [S_Y7]
  Data Type Conversion11/1 -> [S_Y8]
  Data Type Conversion12/1 -> [S_G1]
  Data Type Conversion10/1 -> [S_G2]
  Demux13/15 -> Data Type Conversion13/1
  Demux13/13 -> Data Type Conversion14/1
  Demux13/12 -> Data Type Conversion17/1
  Demux13/11 -> Data Type Conversion16/1
  Demux13/14 -> Data Type Conversion15/1
  Data Type Conversion16/1 -> [F3]
  Data Type Conversion17/1 -> [F5]
  Data Type Conversion14/1 -> [F6]
  Data Type Conversion15/1 -> [F7]
  Data Type Conversion13/1 -> [Manual_Reset]
  Data Type Conversion18/1 -> [Grid_enable]
  Demux13/16 -> Data Type Conversion18/1
  Mux17/1 -> Mux3/10
  Mux16/1 -> Mux3/9
  [S_G1] -> Mux16/1
  [S_G2] -> Mux17/1
  Analog outputs init values3/1 -> OpDNP3_AsyncSlaveCtrl1/3
  Analog outputs init values4/1 -> OpDNP3_AsyncSlaveCtrl1/2, OpDNP3_AsyncSlaveCtrl1/4
  Mux13/1 -> OpDNP3_AsyncSlaveCtrl1/1
  OpDNP3_AsyncSlaveCtrl1/2 -> Demux14/1
  Demux14/1 -> [G1_En]
  Demux14/2 -> [Gen_P]
  [S_Gen1] -> Mux13/1
  [Omega_V2] -> Gain6/1
  [Pe2] -> 2 kHz1/1
  [Q2] -> 2 kHz2/1
  Gain2/1 -> Mux13/2
  Gain4/1 -> Mux13/3
  [V2] -> 2 kHz5/1
  Gain6/1 -> Mux13/5
  Demux14/4 -> [Gen_F]
  Demux14/5 -> [Gen_V]
  Demux3/16 -> Goto72/1
  Demux3/15 -> Goto81/1
  Demux3/14 -> Goto80/1
  Demux3/1 -> Goto75/1
  Demux3/2 -> Goto76/1
  Demux3/3 -> Goto58/1
  Demux3/4 -> Goto59/1
  Demux3/5 -> Goto66/1
  Demux3/6 -> Goto67/1
  Demux3/7 -> Goto74/1
  Demux3/8 -> Goto78/1
  Demux3/9 -> Goto73/1
  Demux3/10 -> Goto77/1
  Demux3/11 -> Goto1/1
  Demux3/12 -> Goto9/1
  Demux3/13 -> Goto79/1
  Step1/1 -> Goto70/1
  Constant3/1 -> Goto82/1
  2 kHz1/1 -> Gain2/1
  2 kHz2/1 -> Gain4/1
  Data Type Conversion/1 -> Mux1/3
  2 kHz5/1 -> Mux13/4
  Mux2/1 -> Memory1/1
  [Iabc_BESS2] -> Mux2/6
  connections:
  Load Flow Bus/LConn1 -- Y6/LConn1
  Load Flow Bus/LConn2 -- Y6/LConn2
  Y6/LConn3 -- Load Flow Bus/LConn3
  Load Flow Bus20/RConn1 -- Three-Phase Series RLC Branch21/LConn1 -- Three-Phase Series RLC Branch12/LConn1 -- VI_Y8L/LConn1
  Three-Phase Series RLC Branch12/LConn2 -- VI_Y8L/LConn2 -- Three-Phase Series RLC Branch21/LConn2 -- Load Flow Bus20/RConn2
  VI_Y8L/LConn3 -- Three-Phase Series RLC Branch21/LConn3 -- Load Flow Bus20/RConn3 -- Three-Phase Series RLC Branch12/LConn3
  VI_Y2L1/LConn1 -- Load Flow Bus31/RConn1 -- Distribution XFMR 7/LConn1
  VI_Y2L1/LConn2 -- Distribution XFMR 7/LConn2 -- Load Flow Bus31/RConn2
  Load Flow Bus31/RConn3 -- VI_Y2L1/LConn3 -- Distribution XFMR 7/LConn3
  Distribution XFMR 8/LConn1 -- Three-Phase Series RLC Branch15/LConn3 -- Load Flow Bus44/RConn3
  Load Flow Bus44/RConn2 -- Three-Phase Series RLC Branch15/LConn2 -- Distribution XFMR 8/LConn2
  Distribution XFMR 8/LConn3 -- Three-Phase Series RLC Branch15/LConn1 -- Load Flow Bus44/RConn1
  Distribution XFMR 5/LConn1 -- Three-Phase Series RLC Branch20/LConn1 -- Load Flow Bus66/RConn1
  Load Flow Bus66/RConn2 -- Three-Phase Series RLC Branch20/LConn2 -- Distribution XFMR 5/LConn2
  Load Flow Bus66/RConn3 -- Distribution XFMR 5/LConn3 -- Three-Phase Series RLC Branch20/LConn3
  Three-Phase Series RLC Branch19/LConn1 -- Subsystem4/LConn1 -- Load Flow Bus67/RConn1 -- Distribution XFMR 10/LConn1
  Three-Phase Series RLC Branch19/LConn2 -- Subsystem4/LConn2 -- Load Flow Bus67/RConn2 -- Distribution XFMR 10/LConn2
  VI_Y3R1/RConn1 -- VI_BESS2/LConn1 -- Y2/RConn1 -- Distribution XFMR 6/LConn1
  VI_Y3R1/RConn2 -- VI_BESS2/LConn2 -- Y2/RConn2 -- Distribution XFMR 6/LConn2
  VI_Y3R1/RConn3 -- VI_BESS2/LConn3 -- Y2/RConn3 -- Distribution XFMR 6/LConn3
  Load Flow Bus69/RConn3 -- SSN Interface Block (3ph)1/LConn3 -- Distribution XFMR 3/LConn3
  VI_Y4R1/LConn1 -- VI_Y4R2/RConn1 -- VI_Y4R/RConn1
  VI_Y4R/RConn2 -- VI_Y4R2/RConn2 -- VI_Y4R1/LConn2
  VI_Y4R1/LConn3 -- VI_Y4R2/RConn3 -- VI_Y4R/RConn3
  Distribution XFMR 02/LConn1 -- StubLine/LConn1 -- Three-Phase Series RLC Branch1/LConn1 -- Subsystem/LConn1 -- Load Flow Bus36/RConn1
  Distribution XFMR 04/LConn1 -- StubLine1/LConn1 -- Three-Phase Series RLC Branch1/LConn3 -- Subsystem/LConn3 -- Load Flow Bus36/RConn3
  VI_PV1/RConn3 -- SSN Interface Block (3ph)6/RConn3 -- Three-Phase Series RLC Branch9/LConn3
  Triplex 2/RConn1 -- Distribution XFMR 02/RConn2 -- Distribution XFMR 02/LConn2 -- Ground3/LConn1
  Triplex 3/RConn1 -- Distribution XFMR 03/RConn2 -- Ground4/LConn1 -- Distribution XFMR 03/LConn2
  Triplex 4/RConn1 -- Distribution XFMR 04/RConn2 -- Ground/LConn1 -- Distribution XFMR 04/LConn2
  Distribution XFMR 05/RConn2 -- Triplex 5/RConn1 -- Ground2/LConn1 -- Distribution XFMR 05/LConn2
  Three-Phase Series RLC Branch22/LConn1 -- Three-Phase Series RLC Branch11/LConn1 -- VI_Y5R/RConn1 -- Distribution XFMR 4/LConn1
  Three-Phase Series RLC Branch22/LConn2 -- Three-Phase Series RLC Branch11/LConn2 -- VI_Y5R/RConn2 -- Distribution XFMR 4/LConn2
  VI_Y5R/RConn3 -- Distribution XFMR 4/LConn3 -- Three-Phase Series RLC Branch22/LConn3 -- Three-Phase Series RLC Branch11/LConn3
  Distribution XFMR 07/LConn1 -- Three-Phase Series RLC Branch24/LConn1 -- Load Flow Bus49/RConn1
  Distribution XFMR 07/LConn2 -- Three-Phase Series RLC Branch24/LConn2 -- Load Flow Bus49/RConn2
  Load Flow Bus49/RConn3 -- Three-Phase Series RLC Branch24/LConn3 -- Distribution XFMR 07/LConn3
  Distribution XFMR 09/LConn1 -- Subsystem3/LConn1 -- Three-Phase Series RLC Branch26/LConn1 -- Load Flow Bus53/RConn1
  Distribution XFMR 09/LConn2 -- Subsystem3/LConn2 -- Three-Phase Series RLC Branch26/LConn2 -- Load Flow Bus53/RConn2
  Distribution XFMR 09/LConn3 -- Subsystem3/LConn3 -- Three-Phase Series RLC Branch26/LConn3 -- Load Flow Bus53/RConn3
  VI_Y6R/RConn2 -- Three-Phase Series RLC Branch28/LConn2 -- Distribution XFMR 011/LConn2
  VI_Y6R/RConn1 -- Three-Phase Series RLC Branch28/LConn1 -- Distribution XFMR 011/LConn1
  VI_Y6R/RConn3 -- Three-Phase Series RLC Branch28/LConn3 -- Distribution XFMR 011/LConn3
  Distribution XFMR 013/LConn1 -- Subsystem2/LConn1 -- Three-Phase Series RLC Branch30/LConn1 -- Load Flow Bus60/RConn1
  Load Flow Bus60/RConn2 -- Subsystem2/LConn2 -- Three-Phase Series RLC Branch30/LConn2 -- Distribution XFMR 013/LConn2
  Load Flow Bus60/RConn3 -- Subsystem2/LConn3 -- Three-Phase Series RLC Branch30/LConn3 -- Distribution XFMR 013/LConn3
  VI_PV1/RConn2 -- SSN Interface Block (3ph)6/RConn2 -- Three-Phase Series RLC Branch9/LConn2
  Three-Phase Series RLC Branch9/LConn1 -- SSN Interface Block (3ph)6/RConn1 -- VI_PV1/RConn1
  Load Flow Bus69/RConn1 -- SSN Interface Block (3ph)1/LConn1 -- Distribution XFMR 3/LConn1
  Three-Phase Series RLC Branch19/LConn3 -- Subsystem4/LConn3 -- Load Flow Bus67/RConn3 -- Distribution XFMR 10/LConn3
  Load Flow Bus65/RConn1 -- Distribution XFMR 014/RConn1
  Load Flow Bus62/RConn2 -- Distribution XFMR 011/RConn2
  Three-Phase Series RLC Branch24/RConn2 -- Load Flow Bus50/LConn2
  Load Flow Bus64/LConn3 -- Triplex 13/LConn3
  Three-Phase Series RLC Branch28/RConn3 -- Load Flow Bus59/LConn3
  Three-Phase Series RLC Branch24/RConn1 -- Load Flow Bus50/LConn1
  Three-Phase Series RLC Branch27/RConn1 -- Load Flow Bus58/LConn1
  Load Flow Bus62/LConn1 -- Triplex 11/LConn1
  Load Flow Bus57/LConn2 -- Triplex 10/LConn2
  Load Flow Bus38/LConn3 -- VI_Y7R1/RConn3
  Distribution XFMR 014/LConn2 -- Load Flow Bus61/RConn2
  Load Flow Bus52/LConn1 -- Triplex 8/LConn1
  Three-Phase Series RLC Branch28/RConn2 -- Load Flow Bus59/LConn2
  Three-Phase Series RLC Branch25/RConn1 -- Load Flow Bus53/LConn1
  Load Flow Bus54/RConn2 -- Distribution XFMR 010/LConn2
  Load Flow Bus57/RConn2 -- Distribution XFMR 010/RConn2
  VI_BESS4/RConn1 -- Three-Phase Series RLC Branch17/LConn1
  Distribution XFMR 09/RConn2 -- Load Flow Bus56/RConn2
  Load Flow Bus57/RConn1 -- Distribution XFMR 010/RConn1
  Load Flow Bus56/LConn2 -- Triplex 9/LConn2
  Three-Phase Series RLC Branch26/RConn2 -- Load Flow Bus54/LConn2
  Three-Phase Series RLC Branch27/RConn2 -- Load Flow Bus58/LConn2
  Distribution XFMR 08/LConn3 -- Load Flow Bus50/RConn3
  Distribution XFMR 014/LConn3 -- Load Flow Bus61/RConn3
  PV Farm 2 MW1/RConn1 -- Three-Phase Series RLC Branch18/LConn1
  Three-Phase Series RLC Branch13/LConn3 -- Load 15/LConn3 -- Load Flow Bus/RConn3
  Distribution XFMR 014/LConn1 -- Load Flow Bus61/RConn1
  Three-Phase Series RLC Branch18/RConn1 -- Y16/LConn1
  Y12/LConn1 -- VI_Y7R1/LConn1
  Three-Phase Series RLC Branch18/LConn2 -- PV Farm 2 MW1/RConn2
  Three-Phase Transformer (Two Windings)/LConn1 -- Y4/LConn1
  "Battery 1 "/RConn3 -- Three-Phase Series RLC Branch16/RConn3
  VI_BESS2/RConn1 -- Y20/LConn1
  Y12/LConn3 -- VI_Y7R1/LConn3
  Three-Phase Series RLC Branch18/RConn3 -- Y16/LConn3
  Three-Phase Transformer (Two Windings)/RConn1 -- VI_BESS6/LConn1
  VI_BESS4/RConn3 -- Three-Phase Series RLC Branch17/LConn3
  Distribution XFMR 1/LConn1 -- Y4/RConn1 -- Y1/LConn1 -- SSN Interface Block (3ph)6/LConn1 -- Load Flow Bus38/RConn1
  VI_PV1/LConn3 -- Y16/RConn3
  VI_BESS4/LConn1 -- Three-Phase Transformer (Two Windings)2/RConn1
  Three-Phase Series RLC Branch26/RConn3 -- Load Flow Bus54/LConn3
  Load Flow Bus51/RConn2 -- Distribution XFMR 07/RConn2
  Three-Phase Series RLC Branch26/RConn1 -- Load Flow Bus54/LConn1
  Y21/LConn1 -- VI_Y1R1/LConn1
  Three-Phase Series RLC Branch29/RConn3 -- Load Flow Bus60/LConn3
  Distribution XFMR 1/LConn3 -- Y4/RConn3 -- Y1/LConn3 -- SSN Interface Block (3ph)6/LConn3 -- Load Flow Bus38/RConn3
  Load Flow Bus38/LConn2 -- VI_Y7R1/RConn2
  Battery 2/RConn1 -- Three-Phase Series RLC Branch17/RConn1
  "Battery 1 "/RConn2 -- Three-Phase Series RLC Branch16/RConn2
  Distribution XFMR 09/RConn1 -- Load Flow Bus56/RConn1
  Three-Phase Series RLC Branch13/LConn1 -- Load 15/LConn1 -- Load Flow Bus/RConn1
  VI_BESS2/RConn3 -- Y20/LConn3
  Y21/LConn3 -- VI_Y1R1/LConn3
  Three-Phase Series RLC Branch30/RConn1 -- Load Flow Bus61/LConn1
  Load Flow Bus57/RConn3 -- Distribution XFMR 010/RConn3
  Three-Phase Series RLC Branch28/RConn1 -- Load Flow Bus59/LConn1
  Three-Phase Series RLC Branch17/RConn2 -- Battery 2/RConn2
  Three-Phase Series RLC Branch29/RConn2 -- Load Flow Bus60/LConn2
  Three-Phase Series RLC Branch27/RConn3 -- Load Flow Bus58/LConn3
  Load Flow Bus52/LConn2 -- Triplex 8/LConn2
  Y21/RConn1 -- VI_Y1L1/RConn1
  Three-Phase Series RLC Branch30/RConn2 -- Load Flow Bus61/LConn2
  PV Farm 2 MW1/RConn3 -- Three-Phase Series RLC Branch18/LConn3
  Three-Phase Transformer (Two Windings)/LConn2 -- Y4/LConn2
  Three-Phase Series RLC Branch18/RConn2 -- Y16/LConn2
  VI_BESS2/RConn2 -- Y20/LConn2
  Three-Phase Transformer (Two Windings)2/LConn3 -- Y20/RConn3
  Load Flow Bus38/RConn2 -- Y4/RConn2 -- Y1/LConn2 -- SSN Interface Block (3ph)6/LConn2 -- Distribution XFMR 1/LConn2
  Load Flow Bus56/LConn1 -- Triplex 9/LConn1
  Y12/RConn2 -- VI_Y7L1/RConn2
  Three-Phase Transformer (Two Windings)/RConn2 -- VI_BESS6/LConn2
  "Battery 1 "/RConn1 -- Three-Phase Series RLC Branch16/RConn1
  Load Flow Bus38/LConn1 -- VI_Y7R1/RConn1
  Three-Phase Transformer (Two Windings)/RConn3 -- VI_BESS6/LConn3
  VI_PV1/LConn1 -- Y16/RConn1
  VI_PV1/LConn2 -- Y16/RConn2
  Three-Phase Transformer (Two Windings)/LConn3 -- Y4/LConn3
  VI_BESS4/LConn3 -- Three-Phase Transformer (Two Windings)2/RConn3
  Three-Phase Transformer (Two Windings)2/LConn2 -- Y20/RConn2
  Three-Phase Series RLC Branch17/RConn3 -- Battery 2/RConn3
  Y12/RConn1 -- VI_Y7L1/RConn1
  Three-Phase Series RLC Branch13/LConn2 -- Load 15/LConn2 -- Load Flow Bus/RConn2
  VI_BESS4/LConn2 -- Three-Phase Transformer (Two Windings)2/RConn2
  SSN Interface Block (3ph)4/LConn1 -- Load Flow Bus37/RConn1 -- Distribution XFMR 14/LConn1
  Three-Phase Series RLC Branch/RConn1 -- VI_Y7L1/LConn1
  VI_BESS4/RConn2 -- Three-Phase Series RLC Branch17/LConn2
  Three-Phase Series RLC Branch/RConn2 -- VI_Y7L1/LConn2
  Three-Phase Series RLC Branch/RConn3 -- VI_Y7L1/LConn3
  Three-Phase Series RLC Branch29/LConn1 -- SSN Interface Block (3ph)3/RConn1 -- Distribution XFMR 012/LConn1
  Three-Phase Series RLC Branch29/LConn2 -- Distribution XFMR 012/LConn2 -- SSN Interface Block (3ph)3/RConn2
  Distribution XFMR 14/LConn2 -- SSN Interface Block (3ph)4/LConn2 -- Load Flow Bus37/RConn2
  Three-Phase Transformer (Two Windings)2/LConn1 -- Y20/RConn1
  SSN Interface Block (3ph)4/LConn3 -- Load Flow Bus37/RConn3 -- Distribution XFMR 14/LConn3
  Three-Phase Series RLC Branch29/LConn3 -- Distribution XFMR 012/LConn3 -- SSN Interface Block (3ph)3/RConn3
  VI_Y3L1/LConn3 -- Load Flow Bus68/RConn3
  Three-Phase Series RLC Branch4/RConn3 -- Load Flow Bus69/LConn3
  Load Flow Bus26/LConn2 -- Load 5/LConn2
  Y12/RConn3 -- VI_Y7L1/RConn3
  Y10/RConn1 -- VI_Y6L/RConn1
  VI_Y1R1/RConn1 -- Load Flow Bus20/LConn1
  VI_Y4R/LConn2 -- Y24/LConn2
  Three-Phase Series RLC Branch14/LConn1 -- VI_Y2R1/RConn1
  Y24/RConn2 -- VI_Y4L/RConn2
  Y23/RConn1 -- VI_Y3L1/RConn1
  Y23/RConn2 -- VI_Y3L1/RConn2
  Y22/RConn3 -- VI_Y2L1/RConn3
  Y21/RConn3 -- VI_Y1L1/RConn3
  Three-Phase Series RLC Branch13/RConn1 -- VI_Y1L1/LConn1
  Load Flow Bus26/LConn3 -- Load 5/LConn3
  Y10/RConn2 -- VI_Y6L/RConn2
  Y22/LConn3 -- VI_Y2R1/LConn3
  VI_Y1R1/LConn2 -- Y21/LConn2
  Y22/LConn1 -- VI_Y2R1/LConn1
  VI_Y2R1/LConn2 -- Y22/LConn2
  Y24/RConn3 -- VI_Y4L/RConn3
  VI_Y6L/LConn2 -- Load Flow Bus58/RConn2
  Three-Phase Series RLC Branch20/RConn2 -- Load Flow Bus67/LConn2
  Three-Phase Series RLC Branch19/RConn3 -- Load Flow Bus68/LConn3
  VI_Y6R/LConn2 -- Y10/LConn2
  Load Flow Bus55/RConn2 -- Distribution XFMR 9/LConn2
  Three-Phase Series RLC Branch13/RConn3 -- VI_Y1L1/LConn3
  Y21/RConn2 -- VI_Y1L1/RConn2
  Y25/LConn1 -- VI_Y5R/LConn1
  Y22/RConn2 -- VI_Y2L1/RConn2
  VI_Y5L/LConn3 -- Load Flow Bus43/RConn3
  VI_Y3L1/LConn2 -- Load Flow Bus68/RConn2
  Y23/LConn3 -- VI_Y3R1/LConn3
  VI_Y3L1/LConn1 -- Load Flow Bus68/RConn1
  VI_Y3R1/LConn2 -- Y23/LConn2
  Three-Phase Series RLC Branch13/RConn2 -- VI_Y1L1/LConn2
  Y23/LConn1 -- VI_Y3R1/LConn1
  Y23/RConn3 -- VI_Y3L1/RConn3
  Y24/LConn1 -- VI_Y4R/LConn1
  Three-Phase Series RLC Branch14/LConn3 -- VI_Y2R1/RConn3
  Three-Phase Series RLC Branch14/LConn2 -- VI_Y2R1/RConn2
  VI_Y4L/LConn3 -- Load Flow Bus70/RConn3
  VI_Y1R1/RConn3 -- Load Flow Bus20/LConn3
  Y24/RConn1 -- VI_Y4L/RConn1
  Three-Phase Series RLC Branch3/RConn2 -- Load Flow Bus70/LConn2
  Load Flow Bus27/LConn1 -- Load 10/LConn1
  Load Flow Bus25/LConn1 -- Load 9/LConn1
  Load Flow Bus23/LConn1 -- Load 7/LConn1
  VI_Y1R1/RConn2 -- Load Flow Bus20/LConn2
  Y25/RConn2 -- VI_Y5L/RConn2
  VI_Y4L/LConn1 -- Load Flow Bus70/RConn1
  Three-Phase Series RLC Branch5/RConn2 -- Load Flow Bus21/LConn2
  Three-Phase Series RLC Branch6/RConn3 -- Load Flow Bus22/LConn3
  Distribution XFMR 2/RConn2 -- Load Flow Bus30/RConn2
  Load Flow Bus28/LConn3 -- Load 6/LConn3
  Three-Phase Series RLC Branch4/RConn2 -- Load Flow Bus69/LConn2
  Load Flow Bus32/LConn1 -- Load 11/LConn1
  Three-Phase Series RLC Branch3/RConn1 -- Load Flow Bus70/LConn1
  Load Flow Bus55/RConn1 -- Distribution XFMR 9/LConn1
  Three-Phase Series RLC Branch5/RConn1 -- Load Flow Bus21/LConn1
  Load Flow Bus24/RConn1 -- Distribution XFMR 8/RConn1
  Y10/RConn3 -- VI_Y6L/RConn3
  Load 14/LConn1 -- Load Flow Bus30/LConn1
  VI_Y7R1/LConn2 -- Y12/LConn2
  Three-Phase Series RLC Branch4/RConn1 -- Load Flow Bus69/LConn1
  Y22/RConn1 -- VI_Y2L1/RConn1
  VI_Y6L/LConn3 -- Load Flow Bus58/RConn3
  Three-Phase Series RLC Branch15/RConn1 -- Load Flow Bus55/LConn1
  Load Flow Bus28/LConn2 -- Load 6/LConn2
  Load Flow Bus29/LConn2 -- Load 3/LConn2
  Load Flow Bus26/RConn3 -- Distribution XFMR 5/RConn3
  VI_Y6L/LConn1 -- Load Flow Bus58/RConn1
  Load Flow Bus23/LConn3 -- Load 7/LConn3
  Load Flow Bus27/LConn3 -- Load 10/LConn3
  Y10/LConn3 -- VI_Y6R/LConn3
  VI_Y5L/LConn1 -- Load Flow Bus43/RConn1
  Three-Phase Series RLC Branch6/RConn1 -- Load Flow Bus22/LConn1
  Y24/LConn3 -- VI_Y4R/LConn3
  Y25/RConn3 -- VI_Y5L/RConn3
  Distribution XFMR 12/RConn1 -- Load Flow Bus33/RConn1
  Load Flow Bus55/RConn3 -- Distribution XFMR 9/LConn3
  Load Flow Bus28/RConn2 -- Distribution XFMR 6/RConn2
  Three-Phase Series RLC Branch3/RConn3 -- Load Flow Bus70/LConn3
  VI_Y5R/LConn2 -- Y25/LConn2
  Three-Phase Series RLC Branch19/RConn2 -- Load Flow Bus68/LConn2
  Three-Phase Series RLC Branch15/RConn2 -- Load Flow Bus55/LConn2
  Load Flow Bus29/LConn1 -- Load 3/LConn1
  Distribution XFMR 2/RConn3 -- Load Flow Bus30/RConn3
  Load Flow Bus26/LConn1 -- Load 5/LConn1
  Load Flow Bus27/RConn1 -- Distribution XFMR 10/RConn1
  Three-Phase Series RLC Branch20/RConn3 -- Load Flow Bus67/LConn3
  VI_Y5L/LConn2 -- Load Flow Bus43/RConn2
  Three-Phase Series RLC Branch19/RConn1 -- Load Flow Bus68/LConn1
  Three-Phase Series RLC Branch6/RConn2 -- Load Flow Bus22/LConn2
  Y25/RConn1 -- VI_Y5L/RConn1
  Three-Phase Series RLC Branch15/RConn3 -- Load Flow Bus55/LConn3
  VI_Y4L/LConn2 -- Load Flow Bus70/RConn2
  Load Flow Bus27/LConn2 -- Load 10/LConn2
  Three-Phase Series RLC Branch5/RConn3 -- Load Flow Bus21/LConn3
  Three-Phase Series RLC Branch20/RConn1 -- Load Flow Bus67/LConn1
  Load Flow Bus26/RConn2 -- Distribution XFMR 5/RConn2
  Three-Phase Series RLC Branch1/RConn3 -- Load Flow Bus37/LConn3
  Three-Phase Series RLC Branch1/LConn2 -- Subsystem/LConn2 -- Load Flow Bus36/RConn2
  Distribution XFMR 1/RConn3 -- Load Flow Bus40/RConn3
  Distribution XFMR 12/RConn3 -- Load Flow Bus33/RConn3
  Y25/LConn3 -- VI_Y5R/LConn3
  Y10/LConn1 -- VI_Y6R/LConn1
  Load Flow Bus23/RConn3 -- Distribution XFMR 7/RConn3
  Load Flow Bus32/LConn2 -- Load 11/LConn2
  Load 14/LConn2 -- Load Flow Bus30/LConn2
  Load Flow Bus46/RConn2 -- Distribution XFMR 06/LConn2
  Three-Phase Series RLC Branch23/RConn3 -- Load Flow Bus49/LConn3
  Distribution XFMR 4/RConn1 -- Load Flow Bus45/RConn1
  Load Flow Bus32/LConn3 -- Load 11/LConn3
  Load Flow Bus29/RConn1 -- Distribution XFMR 3/RConn1
  Three-Phase Series RLC Branch10/RConn1 -- Load Flow Bus43/LConn1
  Load Flow Bus32/RConn3 -- Distribution XFMR 11/RConn3
  Load 2/LConn3 -- Load Flow Bus39/LConn3
  Load Flow Bus23/LConn2 -- Load 7/LConn2
  Load Flow Bus52/RConn2 -- Distribution XFMR 08/RConn2
  Three-Phase Series RLC Branch1/RConn1 -- Load Flow Bus37/LConn1
  Load Flow Bus23/RConn2 -- Distribution XFMR 7/RConn2
  Load Flow Bus25/LConn3 -- Load 9/LConn3
  Load Flow Bus24/RConn2 -- Distribution XFMR 8/RConn2
  Load 1/LConn3 -- Load Flow Bus40/LConn3
  Load Flow Bus28/RConn3 -- Distribution XFMR 6/RConn3
  Load Flow Bus46/RConn1 -- Distribution XFMR 06/LConn1
  Three-Phase Series RLC Branch10/RConn2 -- Load Flow Bus43/LConn2
  Load Flow Bus33/RConn2 -- Distribution XFMR 12/RConn2
  Load Flow Bus28/RConn1 -- Distribution XFMR 6/RConn1
  Load Flow Bus27/RConn3 -- Distribution XFMR 10/RConn3
  Three-Phase Series RLC Branch2/RConn2 -- Load Flow Bus36/LConn2
  Load 4/LConn2 -- Load Flow Bus45/LConn2
  Load Flow Bus23/RConn1 -- Distribution XFMR 7/RConn1
  Load Flow Bus24/LConn3 -- Load 8/LConn3
  Load Flow Bus24/LConn1 -- Load 8/LConn1
  Load Flow Bus29/RConn3 -- Distribution XFMR 3/RConn3
  Load Flow Bus24/LConn2 -- Load 8/LConn2
  Three-Phase Series RLC Branch1/RConn2 -- Load Flow Bus37/LConn2
  Load Flow Bus45/RConn2 -- Distribution XFMR 4/RConn2
  Load Flow Bus28/LConn1 -- Load 6/LConn1
  Load Flow Bus29/RConn2 -- Distribution XFMR 3/RConn2
  Distribution XFMR 2/RConn1 -- Load Flow Bus30/RConn1
  Load Flow Bus32/RConn2 -- Distribution XFMR 11/RConn2
  Load 1/LConn1 -- Load Flow Bus40/LConn1
  Load Flow Bus24/RConn3 -- Distribution XFMR 8/RConn3
  Three-Phase Series RLC Branch25/RConn2 -- Load Flow Bus53/LConn2
  Distribution XFMR 08/LConn1 -- Load Flow Bus50/RConn1
  Load Flow Bus25/LConn2 -- Load 9/LConn2
  Load Flow Bus32/RConn1 -- Distribution XFMR 11/RConn1
  Load Flow Bus47/LConn1 -- Triplex 6/LConn1
  Load Flow Bus26/RConn1 -- Distribution XFMR 5/RConn1
  Load Flow Bus25/RConn2 -- Distribution XFMR 9/RConn2
  Load Flow Bus27/RConn2 -- Distribution XFMR 10/RConn2
  Load Flow Bus25/RConn1 -- Distribution XFMR 9/RConn1
  Distribution XFMR 1/RConn2 -- Load Flow Bus40/RConn2
  Distribution XFMR 05/LConn1 -- Load Flow Bus42/RConn1
  Load Flow Bus47/LConn3 -- Triplex 6/LConn3
  Load 14/LConn3 -- Load Flow Bus30/LConn3
  Load Flow Bus25/RConn3 -- Distribution XFMR 9/RConn3
  Load Flow Bus29/LConn3 -- Load 3/LConn3
  StubLine1/RConn1 -- Load Flow Bus42/LConn1
  Triplex 5/LConn1 -- Distribution XFMR 05/RConn1
  Three-Phase Series RLC Branch24/RConn3 -- Load Flow Bus50/LConn3
  Three-Phase Series RLC Branch23/RConn1 -- Load Flow Bus49/LConn1
  Load Flow Bus51/RConn1 -- Distribution XFMR 07/RConn1
  Load Flow Bus62/RConn3 -- Distribution XFMR 011/RConn3
  Load Flow Bus52/LConn3 -- Triplex 8/LConn3
  Distribution XFMR 1/RConn1 -- Load Flow Bus40/RConn1
  Load Flow Bus51/LConn2 -- Triplex 7/LConn2
  Distribution XFMR 08/LConn2 -- Load Flow Bus50/RConn2
  Load Flow Bus64/RConn3 -- Distribution XFMR 013/RConn3
  Load Flow Bus65/LConn2 -- Triplex 14/LConn2
  Three-Phase Series RLC Branch2/RConn3 -- Load Flow Bus36/LConn3
  Load Flow Bus47/RConn1 -- Distribution XFMR 06/RConn1
  Load Flow Bus54/RConn3 -- Distribution XFMR 010/LConn3
  Load Flow Bus57/LConn1 -- Triplex 10/LConn1
  Load Flow Bus63/LConn3 -- Triplex 12/LConn3
  Load Flow Bus65/RConn3 -- Distribution XFMR 014/RConn3
  Load Flow Bus51/RConn3 -- Distribution XFMR 07/RConn3
  Load Flow Bus47/RConn2 -- Distribution XFMR 06/RConn2
  Load Flow Bus39/RConn2 -- Distribution XFMR 14/RConn2
  Load Flow Bus39/RConn3 -- Distribution XFMR 14/RConn3
  Load Flow Bus65/RConn2 -- Distribution XFMR 014/RConn2
  Distribution XFMR 4/RConn3 -- Load Flow Bus45/RConn3
  Three-Phase Series RLC Branch30/RConn3 -- Load Flow Bus61/LConn3
  Load 4/LConn3 -- Load Flow Bus45/LConn3
  Load Flow Bus46/RConn3 -- Distribution XFMR 06/LConn3
  Load Flow Bus39/RConn1 -- Distribution XFMR 14/RConn1
  Load Flow Bus52/RConn3 -- Distribution XFMR 08/RConn3
  Three-Phase Series RLC Branch23/RConn2 -- Load Flow Bus49/LConn2
  Load Flow Bus51/LConn3 -- Triplex 7/LConn3
  Load 2/LConn1 -- Load Flow Bus39/LConn1
  Load Flow Bus57/LConn3 -- Triplex 10/LConn3
  Load 2/LConn2 -- Load Flow Bus39/LConn2
  Load Flow Bus65/LConn3 -- Triplex 14/LConn3
  Load Flow Bus63/LConn2 -- Triplex 12/LConn2
  Load Flow Bus47/RConn3 -- Distribution XFMR 06/RConn3
  Load Flow Bus62/LConn3 -- Triplex 11/LConn3
  Load Flow Bus63/RConn2 -- Distribution XFMR 012/RConn2
  Load 4/LConn1 -- Load Flow Bus45/LConn1
  Three-Phase Series RLC Branch11/RConn1 -- Load Flow Bus46/LConn1
  Three-Phase Series RLC Branch2/RConn1 -- Load Flow Bus36/LConn1
  Distribution XFMR 03/LConn1 -- Load Flow Bus41/RConn1
  Three-Phase Series RLC Branch11/RConn2 -- Load Flow Bus46/LConn2
  Three-Phase Series RLC Branch11/RConn3 -- Load Flow Bus46/LConn3
  Triplex 4/LConn1 -- Distribution XFMR 04/RConn1
  Three-Phase Series RLC Branch10/RConn3 -- Load Flow Bus43/LConn3
  Load Flow Bus51/LConn1 -- Triplex 7/LConn1
  Load 1/LConn2 -- Load Flow Bus40/LConn2
  Load Flow Bus47/LConn2 -- Triplex 6/LConn2
  StubLine/RConn1 -- Load Flow Bus41/LConn1
  Load Flow Bus52/RConn1 -- Distribution XFMR 08/RConn1
  Triplex 2/LConn1 -- Distribution XFMR 02/RConn1
  Distribution XFMR 09/RConn3 -- Load Flow Bus56/RConn3
  Distribution XFMR 03/RConn1 -- Triplex 3/LConn1
  Load Flow Bus54/RConn1 -- Distribution XFMR 010/LConn1
  Load Flow Bus62/LConn2 -- Triplex 11/LConn2
  Load Flow Bus62/RConn1 -- Distribution XFMR 011/RConn1
  Load Flow Bus63/RConn3 -- Distribution XFMR 012/RConn3
  Load Flow Bus56/LConn3 -- Triplex 9/LConn3
  Three-Phase Series RLC Branch29/RConn1 -- Load Flow Bus60/LConn1
  Three-Phase Series RLC Branch25/RConn3 -- Load Flow Bus53/LConn3
  Load Flow Bus65/LConn1 -- Triplex 14/LConn1
  Distribution XFMR 012/RConn1 -- Load Flow Bus63/RConn1
  Load Flow Bus63/LConn1 -- Triplex 12/LConn1
  Distribution XFMR 013/RConn2 -- Load Flow Bus64/RConn2
  Distribution XFMR 013/RConn1 -- Load Flow Bus64/RConn1
  Load Flow Bus64/LConn1 -- Triplex 13/LConn1
  Load Flow Bus64/LConn2 -- Triplex 13/LConn2
  Three-Phase Series RLC Branch16/LConn1 -- VI_BESS6/RConn1
  Three-Phase Series RLC Branch16/LConn2 -- VI_BESS6/RConn2
  Three-Phase Series RLC Branch16/LConn3 -- VI_BESS6/RConn3
  Y1/RConn1 -- Three-Phase Transformer (Two Windings)4/RConn1
  Y1/RConn2 -- Three-Phase Transformer (Two Windings)4/RConn2
  Y1/RConn3 -- Three-Phase Transformer (Two Windings)4/RConn3
  Y2/LConn1 -- Three-Phase Transformer (Two Windings)3/RConn3
  Y2/LConn2 -- Three-Phase Transformer (Two Windings)3/RConn2
  Y2/LConn3 -- Three-Phase Transformer (Two Windings)3/RConn1
  VI_Y8R/LConn3 -- Y3/LConn3
  Y3/RConn2 -- VI_Y8L/RConn2
  Y3/RConn3 -- VI_Y8L/RConn3
  VI_Y8R/LConn1 -- Y3/LConn1
  VI_Y8R/LConn2 -- Y3/LConn2
  Y3/RConn1 -- VI_Y8L/RConn1
  Three-Phase Series RLC Branch4/LConn3 -- VI_Y8R/RConn3
  Three-Phase Series RLC Branch4/LConn2 -- VI_Y8R/RConn2
  Three-Phase Series RLC Branch4/LConn1 -- VI_Y8R/RConn1
  V1/LConn1 -- V3/LConn1 -- V2/LConn1
  Y5/RConn1 -- Gen bus/LConn1
  Y5/RConn2 -- Gen bus/LConn2
  Y5/RConn3 -- Gen bus/LConn3
  SSN Interface Block (3ph)4/RConn1 -- Three-Phase Series RLC Branch/LConn1
  SSN Interface Block (3ph)4/RConn2 -- Three-Phase Series RLC Branch/LConn2
  SSN Interface Block (3ph)4/RConn3 -- Three-Phase Series RLC Branch/LConn3
  Three-Phase Series RLC Branch9/RConn1 -- Gen bus/RConn1
  Three-Phase Series RLC Branch9/RConn2 -- Gen bus/RConn2
  Three-Phase Series RLC Branch9/RConn3 -- Gen bus/RConn3
  Gen bus1/RConn1 -- Y5/LConn1
  Gen bus1/RConn2 -- Y5/LConn2
  Gen bus1/RConn3 -- Y5/LConn3
  Gen bus1/LConn1 -- V1/RConn1
  Gen bus1/LConn2 -- V2/RConn1
  Gen bus1/LConn3 -- V3/RConn1
  Load Flow Bus22/RConn1 -- Subsystem1/LConn1 -- Distribution XFMR 12/LConn1
  Load Flow Bus22/RConn2 -- Subsystem1/LConn2 -- Distribution XFMR 12/LConn2
  Load Flow Bus22/RConn3 -- Distribution XFMR 12/LConn3 -- Subsystem1/LConn3
  Load 12/LConn1 -- Load Flow Bus33/LConn1
  Load 12/LConn2 -- Load Flow Bus33/LConn2
  Load 12/LConn3 -- Load Flow Bus33/LConn3
  VI_Y4R1/RConn1 -- Three-Phase Series RLC Branch5/LConn1
  VI_Y4R1/RConn2 -- Three-Phase Series RLC Branch5/LConn2
  VI_Y4R1/RConn3 -- Three-Phase Series RLC Branch5/LConn3
  Distribution XFMR 2/LConn1 -- VI_Y4R2/LConn1
  Distribution XFMR 2/LConn2 -- VI_Y4R2/LConn2
  Distribution XFMR 2/LConn3 -- VI_Y4R2/LConn3
  Three-Phase Series RLC Branch27/LConn1 -- Three-Phase Series RLC Branch25/LConn1 -- Three-Phase Series RLC Branch23/LConn1 -- Load Flow Bus48/RConn1
  Three-Phase Series RLC Branch27/LConn2 -- Three-Phase Series RLC Branch25/LConn2 -- Three-Phase Series RLC Branch23/LConn2 -- Load Flow Bus48/RConn2
  Three-Phase Series RLC Branch27/LConn3 -- Three-Phase Series RLC Branch25/LConn3 -- Three-Phase Series RLC Branch23/LConn3 -- Load Flow Bus48/RConn3
  Three-Phase Series RLC Branch22/RConn1 -- SSN Interface Block (3ph)2/LConn1
  SSN Interface Block (3ph)2/LConn2 -- Three-Phase Series RLC Branch22/RConn2
  Three-Phase Series RLC Branch22/RConn3 -- SSN Interface Block (3ph)2/LConn3
  SSN Interface Block (3ph)2/RConn1 -- Load Flow Bus48/LConn1
  Load Flow Bus48/LConn2 -- SSN Interface Block (3ph)2/RConn2
  SSN Interface Block (3ph)2/RConn3 -- Load Flow Bus48/LConn3
  SSN Interface Block (3ph)3/LConn1 -- Load Flow Bus59/RConn1
  SSN Interface Block (3ph)3/LConn2 -- Load Flow Bus59/RConn2
  SSN Interface Block (3ph)3/LConn3 -- Load Flow Bus59/RConn3
  Three-Phase Series RLC Branch12/RConn1 -- Load Flow Bus31/LConn1
  Three-Phase Series RLC Branch12/RConn2 -- Load Flow Bus31/LConn2
  Three-Phase Series RLC Branch12/RConn3 -- Load Flow Bus31/LConn3
  Distribution XFMR 11/LConn1 -- Load Flow Bus21/RConn1 -- Three-Phase Series RLC Branch6/LConn1
  Distribution XFMR 11/LConn2 -- Load Flow Bus21/RConn2 -- Three-Phase Series RLC Branch6/LConn2
  Three-Phase Series RLC Branch6/LConn3 -- Load Flow Bus21/RConn3 -- Distribution XFMR 11/LConn3
  Distribution XFMR 3/LConn2 -- SSN Interface Block (3ph)1/LConn2 -- Load Flow Bus69/RConn2
  SSN Interface Block (3ph)1/RConn1 -- Three-Phase Series RLC Branch2/LConn1 -- Three-Phase Series RLC Branch3/LConn1
  Three-Phase Series RLC Branch2/LConn2 -- Three-Phase Series RLC Branch3/LConn2 -- SSN Interface Block (3ph)1/RConn2
  Three-Phase Series RLC Branch2/LConn3 -- Three-Phase Series RLC Branch3/LConn3 -- SSN Interface Block (3ph)1/RConn3
  Three-Phase Series RLC Branch10/LConn1 -- SSN Interface Block (3ph)1/RConn4
  SSN Interface Block (3ph)1/RConn5 -- Three-Phase Series RLC Branch10/LConn2
  SSN Interface Block (3ph)1/RConn6 -- Three-Phase Series RLC Branch10/LConn3
  SSN Interface Block (3ph)5/LConn1 -- Three-Phase Series RLC Branch14/RConn1
  SSN Interface Block (3ph)5/LConn2 -- Three-Phase Series RLC Branch14/RConn2
  SSN Interface Block (3ph)5/LConn3 -- Three-Phase Series RLC Branch14/RConn3
  SSN Interface Block (3ph)5/RConn1 -- Load Flow Bus44/LConn1
  SSN Interface Block (3ph)5/RConn2 -- Load Flow Bus44/LConn2
  SSN Interface Block (3ph)5/RConn3 -- Load Flow Bus44/LConn3
  SSN Interface Block (3ph)7/LConn1 -- Three-Phase Series RLC Branch21/RConn1
  SSN Interface Block (3ph)7/LConn2 -- Three-Phase Series RLC Branch21/RConn2
  SSN Interface Block (3ph)7/LConn3 -- Three-Phase Series RLC Branch21/RConn3
  SSN Interface Block (3ph)7/RConn1 -- Load Flow Bus66/LConn1
  SSN Interface Block (3ph)7/RConn2 -- Load Flow Bus66/LConn2
  SSN Interface Block (3ph)7/RConn3 -- Load Flow Bus66/LConn3
  Substation/RConn1 -- Load 13/LConn1 -- Y6/RConn1
  Substation/RConn2 -- Load 13/LConn2 -- Y6/RConn2
  Substation/RConn3 -- Load 13/LConn3 -- Y6/RConn3
